simulink model "IEEE_34_node_2020a_scenarios"  (R2020a)
settings: Solver=FixedStepDiscrete  StartTime=0.0  StopTime=0.001  RelTol=1e-3
InitFcn:
  | power_34NodeTestFeeder_init;
  | %=============================
  | Vnom_ph_ph = 24900;
  | Vnom = 24900/sqrt(3);
  | Vnom1_ph_ph = 4160;
  | Vnom1 = 4160/sqrt(3);
  | Degrees_ph_ph_gen1 = 0;
  | Frequency = 60;
  | Apparent_power_gen1 = 2500e3;
  | base_current=1.5e6;
  | SW850_816=1;
  | SW818_820=1;
  | SW832_858=1;
  | SW834_842=1;
  | SW836_862=1;
  | %=============================
  | %824-828===Load1=================
  | V_824_828 = [1.008 1.016 1.012];
  | Pa_824_828 = [1e-6 1e-6 4]*1e3*1;
  | Pp_824_828 = [1e-6 1e-6 2]*1e3*1;
  | Pn_824_828 = [1e-6 1e-6 1e-6]*1;
  | 
  | %820-822===Load2=================
  | V_820_822 = 0.993;
  | Pa_820_822 = 135e3*1;
  | Pp_820_822 = 70e3*1;
  | Pn_820_822 = 1e-6*1;
  | 
  | %858-834===Load3=================
  | V_858_834 = [1.034 1.032 1.034]*sqrt(3);
  | Pa_858_834 = [4 15 13]*1e3*1;
  | Pp_858_834 = [2 8 7]*1e3*1;
  | Pn_858_834 = [1e-6 1e-6 1e-6]*1;
  | 
  | %844 B.V.c===Load4================
  | V_844 = [1.031 1.029 1.031];
  | Pa_844 = [135 135 135]*1e3*1;
  | Pp_844 = [105 105 105]*1e3*1;
  | Pn_844 = [100 100 100]*1e3*1;
  | 
  | %840======Load5=================
  | V_840 = [1.03 1.029 1.031];
  | Pa_840 = [9 9 9]*1e3*1;
  | Pp_840 = [7 7 7]*1e3*1;
  | Pn_840 = [1e-6 1e-6 1e-6]*1;
  | 
  | % For Distributed Loads==================================================
  | %802-806
  | V_802_806 = [1.047 1.048 1.048];
  | Pa_802_806 = [1e-6 30 25]*1e3;
  | Pp_802_806 = [1e-6 15 14]*1e3;
  | Pn_802_806 = [1e-6 1e-6 1e-6];
  | 
  | %808-810
  | V_808_810 = 1.014;
  | Pa_808_810 = 16e3;
  | Pp_808_810 = 8e3;
  | Pn_808_810 = 1e-6;
  | 
  | %816-824
  | V_816_824 = [1.017 1.025 1.02]*sqrt(3);
  | Pa_816_824 = [1e-6 5 1e-6]*1e3;
  | Pp_816_824 = [1e-6 2 1e-6]*1e3;
  | Pn_816_824 = [1e-6 1e-6 1e-6];
  | 
  | %818-820
  | V_818_820 = 1.016;
  | Pa_818_820 = 34e3;
  | Pp_818_820 = 17e3;
  | Pn_818_820 = 1e-6;
  | 
  | %824-826
  | V_824_826 = 1.008;
  | Pa_824_826 = 40e3;
  | Pp_824_826 = 20e3;
  | Pn_824_826 = 1e-6;
  | 
  | %828-830
  | V_828_830 = [1.007 1.015 1.011];
  | Pa_828_830 = [7 1e-6 1e-6]*1e3;
  | Pp_828_830 = [3 1e-6 1e-6]*1e3;
  | Pn_828_830 = [1e-6 1e-6 1e-6];
  | 
  | %832-858
  | V_832_858 = [1.036 1.035 1.036]*sqrt(3);
  | Pa_832_858 = [7 2 6]*1e3;
  | Pp_832_858 = [3 1 3]*1e3;
  | Pn_832_858 = [1e-6 1e-6 1e-6];
  | 
  | %834-860
  | V_834_860 = [1.031 1.029 1.031]*sqrt(3);
  | Pa_834_860 = [16 20 110]*1e3;
  | Pp_834_860 = [8 10 55]*1e3;
  | Pn_834_860 = [1e-6 1e-6 1e-6];
  | 
  | %836-840
  | V_836_840 = [1.03 1.029 1.031]*sqrt(3);
  | Pa_836_840 = [18 22 1e-6]*1e3;
  | Pp_836_840 = [9 11 1e-6]*1e3;
  | Pn_836_840 = [1e-6 1e-6 1e-6];
  | 
  | %842-844
  | V_842_844 = [1.031 1.029 1.031];
  | Pa_842_844 = [9 1e-6 1e-6]*1e3;
  | Pp_842_844 = [5 1e-6 1e-6]*1e3;
  | Pn_842_844 = [1e-6 1e-6 1e-6];
  | 
  | %844-846
  | V_844_846 = [1.031 1.029 1.031];
  | Pa_844_846 = [1e-6 25 20]*1e3;
  | Pp_844_846 = [1e-6 12 11]*1e3;
  | Pn_844_846 = [1e-6 1e-6 1e-6];
  | 
  | %846-848
  | V_846_848 = [1.031 1.029 1.031];
  | Pa_846_848 = [1e-6 23 1e-6]*1e3;
  | Pp_846_848 = [1e-6 11 1e-6]*1e3;
  | Pn_846_848 = [1e-6 1e-6 1e-6];
  | 
  | %854-856
  | V_854_856 = 0.998;
  | Pa_854_856 = 4e3;
  | Pp_854_856 = 2e3;
  | Pn_854_856 = 1e-6;
  | 
  | %858-864
  | V_858_864 = 1.034;
  | Pa_858_864 = 2e3;
  | Pp_858_864 = 1e3;
  | Pn_858_864 = 1e-6;
  | 
  | %860-836
  | V_860_836 = [1.03 1.029 1.031]*sqrt(3);
  | Pa_860_836 = [30 10 42]*1e3;
  | Pp_860_836 = [15 6 22]*1e3;
  | Pn_860_836 = [1e-6 1e-6 1e-6];
  | 
  | %862-838
  | V_862_838 = 1.029;
  | Pa_862_838 = 28e3;
  | Pp_862_838 = 14e3;
  | Pn_862_838 = 1e-6;
  | 
  | % For Spot Loads===========================================================
  | %830
  | V_830 = [0.989 0.998 0.994]*sqrt(3);
  | Pa_830 = [10 10 25]*1e3;
  | Pp_830 = [5 5 10]*1e3;
  | Pn_830 = [1e-6 1e-6 1e-6];
  | 
  | %848 B.V.c
  | V_848 = [1.031 1.029 1.031]*sqrt(3);
  | Pa_848 = [20 20 20]*1e3;
  | Pp_848 = [16 16 16]*1e3;
  | Pn_848 = [150 150 150]*1e3;
  | 
  | %860
  | V_860 = [1.03 1.029 1.031];
  | Pa_860 = [20 20 20]*1e3;
  | Pp_860 = [16 16 16]*1e3;
  | Pn_860 = [1e-6 1e-6 1e-6];
  | 
  | %890
  | V_890 = [0.917 0.924 0.918]*sqrt(3);
  | Pa_890 = [150 150 150]*1e3;
  | Pp_890 = [75 75 75]*1e3;
  | Pn_890 = [1e-6 1e-6 1e-6];
undefined symbols (not defined in the file or in its folder): Angle, C_300, C_301, C_302, C_303, C_304, Degrees_ph, ft2km, L_300, L_301, L_302, L_303, L_304, Magnitude, ph, ph_gen1, R_300, R_301, R_302, R_303, R_304, Vnom_ph
libraries: powerlib x177
(part 1 of 2)
settings Model: Creator=liyifu  LastModifiedBy=l4729
settings DataIOCC: ReturnWorkspaceOutputs=off
settings DebuggingCC: ArithmeticOperatorsInVariantConditions=warning
settings SFSimCC: SimUseLocalCustomCode=off  CustomCodeUndefinedFunction=UseInterfaceOnly
settings RTWCC: RTWUseLocalCustomCode=off

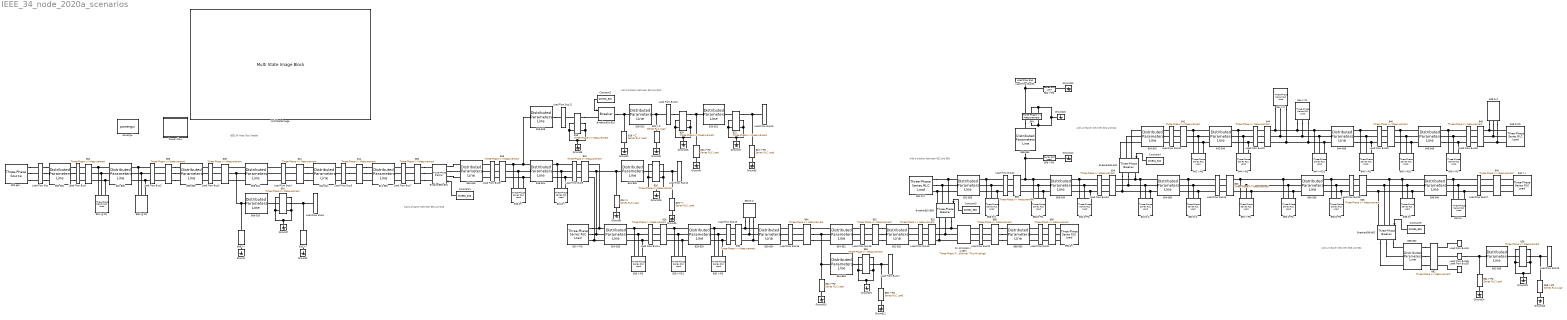
== system IEEE_34_node_2020a_scenarios ==
  note: Add a breaker between 832 and 858.
  note: IEEE 34 Node Test Feeder
  note: Add a breaker between 834 and 842.
  note: Add a breaker between 836 and 862.
  note: Add a breaker between 850 and 816.
  note: Add a breaker between 818 and 820.
  800 gen : powerlib/Electrical Sources/Three-Phase Source  InternalConnection=Yg  VoltagePhases=on  Voltage=Vnom_ph-ph  PhaseAngle=Degrees_ph-ph_gen1  Voltage_phases=[1.05 1.05 1.05]*Vnom  PhaseAngles_phases=[0 -120 +120]  Frequency=Frequency  NonIdealSource=off  SpecifyImpedance=on  Resistance=0.8929  Inductance=16.58e-3  ShortCircuitLevel=Apparent_power_gen1  BaseVoltage=Vnom_ph_ph  XRratio=8  BusType=swing  Pref=10e3  Qref=0  Prefabc=[10e3, 10e3, 10e3]  Qrefabc=[0, 0, 0]  Qmin=-inf  Qmax=inf
  800-802 : powerlib/Elements/Distributed Parameters Line  Phases=3  Frequency=Frequency  Resistance=R_300  Inductance=L_300  Capacitance=C_300  Length=2580*ft2km  x1=[1249.92108084395 26131.4308609001 26009.0181767455;376.991118430775 376.991118430775 376.991118430775;1.94160573810255 0.298080075052811 1.87234868535801]  x2=[1257.88413999223 26107.2604081607 25983.4031146893;376.991118430775 376.991118430775 376.991118430775;1.93808304381954 0.296564583820107 1.87075775483118]  x3=[7.14100156005761 32.3182501048481 23.0835619548769;376.991118430775 376.991118430775 376.991118430775;0.710958188620726 -0.81341186108836 0.253484207816933]  x4=[6.75597430008896 144.846280562991 132.525305942294;376.991118430775 376.991118430775 376.991118430775;-2.867320724315 0.497988283168986 2.04589027410211]  x5=3.46223763231864e-06  V1=ones(3,3)  V2=ones(3,3)  I1=ones(3,3)  I2=ones(3,3)  nHarmo=1  Measurements=None
  802 : powerlib/Measurements/Three-Phase V-I Measurement  VoltageMeasurement=phase-to-ground  SetLabelV=on  LabelV=Vabc_802  Vpu=on  VpuLL=off  CurrentMeasurement=yes  SetLabelI=on  LabelI=Iabc_802  Ipu=on  Pbase=base_current  Vbase=Vnom_ph_ph  OutputType=Magnitude-Angle  PhasorSimulation=on  PSBequivalent=0
  802 Yg PQ : powerlib/Elements/Three-Phase Series RLC Load  LConnTagsString=A|B|C  Configuration=Y (grounded)  NominalVoltage=[  Vabc=V_802_806*Vnom  Vabcp=[1e3 1e3 1e3]  NominalFrequency=Frequency  UnbalancedPower=on  ActivePower=10e3  InductivePower=100  CapacitivePower=100  Pabc=Pa_802_806/2  QLabc=Pp_802_806/2  QCabc=Pn_802_806  Pabcp=[10e3 9e3 11e3]  QLabcp=[100 90 110]  QCabcp=[100 90 110]  Measurements=None  LoadType=constant PQ
      settings: AttributesFormatString=|
      | P= %<Pabc> W
      | Ql=%<QLabc> var
      | Qc=%<QCabc> var
  802-806 : powerlib/Elements/Distributed Parameters Line  Phases=3  Frequency=Frequency  Resistance=R_300  Inductance=L_300  Capacitance=C_300  Length=1730*ft2km  x1=[1257.88413999223 26107.2604081607 25983.4031146893;376.991118430775 376.991118430775 376.991118430775;1.93851306238997 0.296931084446931 1.87111711923874]  x2=[1263.03152773622 26091.3668630639 25967.0505546349;376.991118430775 376.991118430775 376.991118430775;1.93675476604224 0.29592284444399 1.87004699504629]  x3=[6.74174515393169 32.6757565944536 24.2819591482835;376.991118430775 376.991118430775 376.991118430775;0.818712189904275 -0.791719291330259 0.305405947950471]  x4=[6.06467042248893 143.993748432463 131.480607437597;376.991118430775 376.991118430775 376.991118430775;-2.79230394021469 0.498395409094565 2.05596025477108]  x5=2.32157794725242e-06  V1=ones(3,3)  V2=ones(3,3)  I1=ones(3,3)  I2=ones(3,3)  nHarmo=1  Measurements=None
  806 : powerlib/Measurements/Three-Phase V-I Measurement  VoltageMeasurement=phase-to-ground  SetLabelV=on  LabelV=Vabc_806  Vpu=on  VpuLL=off  CurrentMeasurement=yes  SetLabelI=on  LabelI=Iabc_806  Ipu=on  Pbase=base_current  Vbase=Vnom_ph_ph  OutputType=Magnitude-Angle  PhasorSimulation=on  PSBequivalent=0
  806 Yg PQ : powerlib/Elements/Three-Phase Series RLC Load  LConnTagsString=A|B|C  Configuration=Y (grounded)  NominalVoltage=[  Vabc=V_802_806*Vnom  Vabcp=[1e3 1e3 1e3]  NominalFrequency=Frequency  UnbalancedPower=on  ActivePower=10e3  InductivePower=100  CapacitivePower=100  Pabc=Pa_802_806/2  QLabc=Pp_802_806/2  QCabc=Pn_802_806  Pabcp=[10e3 9e3 11e3]  QLabcp=[100 90 110]  QCabcp=[100 90 110]  Measurements=None  LoadType=constant PQ
      settings: AttributesFormatString=|
      | P= %<Pabc> W
      | Ql=%<QLabc> var
      | Qc=%<QCabc> var
  806-808 : powerlib/Elements/Distributed Parameters Line  Phases=3  Frequency=Frequency  Resistance=R_300  Inductance=L_300  Capacitance=C_300  Length=32230*ft2km  x1=[1263.03152773622 26091.3668630639 25967.0505546349;376.991118430775 376.991118430775 376.991118430775;1.9213246879271 0.282771939599148 1.85715215453986]  x2=[1355.36741013163 25802.965279815 25680.3228944133;376.991118430775 376.991118430775 376.991118430775;1.90106006488918 0.264077284558239 1.83705579461531]  x3=[6.38688498732981 32.5400387220186 25.3091222711061;376.991118430775 376.991118430775 376.991118430775;0.921699027337811 -0.793519160961749 0.32962763678599]  x4=[5.32362115475156 140.079806740904 128.071939191277;376.991118430775 376.991118430775 376.991118430775;-2.73237240417034 0.470552224502591 2.03887968104344]  x5=4.32511313525697e-05  V1=ones(3,3)  V2=ones(3,3)  I1=ones(3,3)  I2=ones(3,3)  nHarmo=1  Measurements=None
  808 : powerlib/Measurements/Three-Phase V-I Measurement  VoltageMeasurement=phase-to-ground  SetLabelV=on  LabelV=Vabc_808  Vpu=on  VpuLL=off  CurrentMeasurement=yes  SetLabelI=on  LabelI=Iabc_808  Ipu=on  Pbase=base_current  Vbase=Vnom_ph_ph  OutputType=Magnitude-Angle  PhasorSimulation=on  PSBequivalent=0
  808 Y-I : powerlib/Elements/Series RLC Load  LConnTagsString=a  RConnTagsString=__new0  NominalVoltage=V_808_810*Vnom  NominalFrequency=Frequency  ActivePower=Pa_808_810/2  InductivePower=Pp_808_810/2  CapacitivePower=Pn_808_810  Setx0=off  InitialVoltage=0  SetiL0=off  InitialCurrent=0  Measurements=None  LoadType=constant I
      settings: AttributesFormatString=|
      | P=%<ActivePower> W
      | Ql=%<InductivePower> var
      | Qc=%<CapacitivePower> var
  808-810 : powerlib/Elements/Distributed Parameters Line  Phases=1  Frequency=Frequency  Resistance=R_303(2,2)  Inductance=L_303(2,2)  Capacitance=C_303(2,2)  Length=5804*ft2km  x1=[21046.9259463273;376.991118430775;-2.12176175592429]  x2=[21043.9208768996;376.991118430775;-2.12177244967677]  x3=[34.5685211736535;376.991118430775;-2.11315216164077]  x4=[36.1447450908434;376.991118430775;-2.13270369941523]  x5=7.30496713110932e-06  V1=ones(3,3)  V2=ones(3,3)  I1=ones(3,3)  I2=ones(3,3)  nHarmo=1  Measurements=None
  808-812 : powerlib/Elements/Distributed Parameters Line  Phases=3  Frequency=Frequency  Resistance=R_300  Inductance=L_300  Capacitance=C_300  Length=37500*ft2km  x1=[1355.36741013163 25802.965279815 25680.3228944133;376.991118430775 376.991118430775 376.991118430775;1.89839394975256 0.261804980671934 1.83482773528846]  x2=[1443.84439604931 25478.3634476897 25362.7536549307;376.991118430775 376.991118430775 376.991118430775;1.88315754512085 0.240205062784278 1.81096458108983]  x3=[5.47970534503738 32.5458510221011 26.6156539334698;376.991118430775 376.991118430775 376.991118430775;0.996384506820799 -0.794758877830925 0.308471950569626]  x4=[4.24120551746674 137.246147529385 126.440066991532;376.991118430775 376.991118430775 376.991118430775;-2.80340516655793 0.448617182172184 2.02664641407674]  x5=5.03232213999802e-05  V1=ones(3,3)  V2=ones(3,3)  I1=ones(3,3)  I2=ones(3,3)  nHarmo=1  Measurements=None
  810 : powerlib/Measurements/Three-Phase V-I Measurement  VoltageMeasurement=phase-to-ground  SetLabelV=on  LabelV=Vabc_810  Vpu=on  VpuLL=off  CurrentMeasurement=yes  SetLabelI=on  LabelI=Iabc_810  Ipu=on  Pbase=base_current  Vbase=Vnom_ph_ph  OutputType=Magnitude-Angle  PhasorSimulation=on  PSBequivalent=0
  810 Y-I : powerlib/Elements/Series RLC Load  LConnTagsString=a  RConnTagsString=__new0  NominalVoltage=V_808_810*Vnom  NominalFrequency=Frequency  ActivePower=Pa_808_810/2  InductivePower=Pp_808_810/2  CapacitivePower=Pn_808_810  Setx0=off  InitialVoltage=0  SetiL0=off  InitialCurrent=0  Measurements=None  LoadType=constant I
      settings: AttributesFormatString=|
      | P=%<ActivePower> W
      | Ql=%<InductivePower> var
      | Qc=%<CapacitivePower> var
  812 : powerlib/Measurements/Three-Phase V-I Measurement  VoltageMeasurement=phase-to-ground  SetLabelV=on  LabelV=Vabc_812  Vpu=on  VpuLL=off  CurrentMeasurement=yes  SetLabelI=on  LabelI=Iabc_812  Ipu=on  Pbase=base_current  Vbase=Vnom_ph_ph  OutputType=Magnitude-Angle  PhasorSimulation=on  PSBequivalent=0
  812-814 : powerlib/Elements/Distributed Parameters Line  Phases=3  Frequency=Frequency  Resistance=R_300  Inductance=L_300  Capacitance=C_300  Length=29730*ft2km  x1=[1443.84439604931 25478.3634476897 25362.7536549307;376.991118430775 376.991118430775 376.991118430775;1.88708842075871 0.243555309690653 1.81424959455655]  x2=[1513.83129923695 25224.7890628026 25116.826082141;376.991118430775 376.991118430775 376.991118430775;1.87645290964613 0.226315237464506 1.79513044997697]  x3=[5.55063231072111 32.5564691162332 27.1376298044207;376.991118430775 376.991118430775 376.991118430775;1.01612398171474 -0.820636608900659 0.284298301573858]  x4=[4.1999268951778 136.474072334335 125.741278014505;376.991118430775 376.991118430775 376.991118430775;-2.81942996147556 0.43687198855717 2.01560545263332]  x5=3.98962499259043e-05  V1=ones(3,3)  V2=ones(3,3)  I1=ones(3,3)  I2=ones(3,3)  nHarmo=1  Measurements=None
  814 : powerlib/Measurements/Three-Phase V-I Measurement  VoltageMeasurement=phase-to-ground  SetLabelV=on  LabelV=Vabc_814  Vpu=on  VpuLL=off  CurrentMeasurement=yes  SetLabelI=on  LabelI=Iabc_814  Ipu=on  Pbase=base_current  Vbase=Vnom_ph_ph  OutputType=Magnitude-Angle  PhasorSimulation=on  PSBequivalent=0
  814-850 : powerlib/Elements/Distributed Parameters Line  Phases=3  Frequency=Frequency  Resistance=R_301  Inductance=L_301  Capacitance=C_301  Length=10*ft2km  x1=[749.15329467254 25227.0261178494 25140.714564817;376.991118430775 376.991118430775 376.991118430775;-0.62406898031134 0.237616780416975 1.80414776598586]  x2=[749.130082958643 25226.8770754942 25140.5688252729;376.991118430775 376.991118430775 376.991118430775;-0.624045610021532 0.237609694611455 1.80414003880896]  x3=[4.47496846801465 31.8833259534658 28.1266540016917;376.991118430775 376.991118430775 376.991118430775;0.864239655329809 -0.885362952079534 0.234866042830331]  x4=[4.63631302404033 136.170219123993 125.22263936746;376.991118430775 376.991118430775 376.991118430775;-1.91799176304395 0.450265085785532 2.03068759542421]  x5=1.37899021776565e-08  V1=ones(3,3)  V2=ones(3,3)  I1=ones(3,3)  I2=ones(3,3)  nHarmo=1  Measurements=None
  816 : powerlib/Measurements/Three-Phase V-I Measurement  VoltageMeasurement=phase-to-ground  SetLabelV=on  LabelV=Vabc_816  Vpu=on  VpuLL=off  CurrentMeasurement=yes  SetLabelI=on  LabelI=Iabc_816  Ipu=on  Pbase=base_current  Vbase=Vnom_ph_ph  OutputType=Magnitude-Angle  PhasorSimulation=on  PSBequivalent=0
  816 D-I : powerlib/Elements/Three-Phase Series RLC Load  LConnTagsString=A|B|C  Configuration=Delta  NominalVoltage=[  Vabc=[1.017 1.025 1.02]*sqrt(3)*Vnom  Vabcp=V_816_824*Vnom  NominalFrequency=Frequency  UnbalancedPower=on  ActivePower=10e3  InductivePower=100  CapacitivePower=100  Pabc=[0 30 25]*1e3/2  QLabc=[0 15 14]*1e3/2  QCabc=[0 0 0]  Pabcp=Pa_816_824/2  QLabcp=Pp_816_824/2  QCabcp=Pn_816_824  Measurements=None  LoadType=constant I
      settings: AttributesFormatString=|
      | P= %<Pabc> W
      | Ql=%<QLabc> var
      | Qc=%<QCabc> var
  816-818 : powerlib/Elements/Distributed Parameters Line  Phases=1  Frequency=Frequency  Resistance=R_302(1,1)  Inductance=L_302(1,1)  Capacitance=C_302(1,1)  Length=1710*ft2km  x1=[20490.3042148397;376.991118430775;-0.0532544135280046]  x2=[20490.3109594136;376.991118430775;-0.053255033845596]  x3=[34.5169728301595;376.991118430775;-0.0540660920901116]  x4=[34.5169728344743;376.991118430775;-0.0532550338463431]  x5=2.15222153587128e-06  V1=ones(3,3)  V2=ones(3,3)  I1=ones(3,3)  I2=ones(3,3)  nHarmo=1  Measurements=None
  816-824 : powerlib/Elements/Distributed Parameters Line  Phases=3  Frequency=Frequency  Resistance=R_301  Inductance=L_301  Capacitance=C_301  Length=10210*ft2km  x1=[748.410739748618 25222.2511977151 25136.0453810114;376.991118430775 376.991118430775 376.991118430775;-0.628622488455534 0.233068321988764 1.79964654831585]  x2=[724.867335226711 25070.57527146 24988.5436693509;376.991118430775 376.991118430775 376.991118430775;-0.603933885970706 0.225820727896608 1.79171985964701]  x3=[4.47046107178887 31.6153299611701 28.1466881681829;376.991118430775 376.991118430775 376.991118430775;0.861223606040793 -0.892893782392515 0.231267715388187]  x4=[4.61080299055656 134.671592338258 123.966064883203;376.991118430775 376.991118430775 376.991118430775;-1.92687304548077 0.440217730369648 2.02260235021295]  x5=1.40794901233873e-05  V1=ones(3,3)  V2=ones(3,3)  I1=ones(3,3)  I2=ones(3,3)  nHarmo=1  Measurements=None
  818 : powerlib/Measurements/Three-Phase V-I Measurement  VoltageMeasurement=phase-to-ground  SetLabelV=on  LabelV=Vabc_818  Vpu=on  VpuLL=off  CurrentMeasurement=yes  SetLabelI=on  LabelI=Iabc_818  Ipu=on  Pbase=base_current  Vbase=Vnom_ph_ph  OutputType=Magnitude-Angle  PhasorSimulation=on  PSBequivalent=0
  818 Y-Z : powerlib/Elements/Series RLC Load  LConnTagsString=a  RConnTagsString=__new0  NominalVoltage=V_818_820*Vnom  NominalFrequency=Frequency  ActivePower=Pa_818_820/2  InductivePower=Pp_818_820/2  CapacitivePower=Pn_818_820  Setx0=off  InitialVoltage=0  SetiL0=off  InitialCurrent=0  Measurements=None  LoadType=constant Z
      settings: AttributesFormatString=|
      | P=%<ActivePower> W
      | Ql=%<InductivePower> var
      | Qc=%<CapacitivePower> var
  818-820 : powerlib/Elements/Distributed Parameters Line  Phases=1  Frequency=Frequency  Resistance=R_302(1,1)  Inductance=L_302(1,1)  Capacitance=C_302(1,1)  Length=48150*ft2km  x1=[2.78170730011638e-10;376.991118430775;-2.73913993190896]  x2=[2.75226069334982e-10;376.991118430775;-2.713474091581]  x3=[5.39302235223237e-13;376.991118430775;-2.24824250678969]  x4=[4.97303653528767e-13;376.991118430775;3.01000433404245]  x5=6.06020274574283e-05  V1=ones(3,3)  V2=ones(3,3)  I1=ones(3,3)  I2=ones(3,3)  nHarmo=1  Measurements=None
  820 : powerlib/Measurements/Three-Phase V-I Measurement  VoltageMeasurement=phase-to-ground  SetLabelV=on  LabelV=Vabc_820  Vpu=on  VpuLL=off  CurrentMeasurement=yes  SetLabelI=on  LabelI=Iabc_820  Ipu=on  Pbase=base_current  Vbase=Vnom_ph_ph  OutputType=Magnitude-Angle  PhasorSimulation=on  PSBequivalent=0
  820 Y-PQ : powerlib/Elements/Series RLC Load  LConnTagsString=a  RConnTagsString=__new0  NominalVoltage=V_820_822*Vnom  NominalFrequency=Frequency  ActivePower=Pa_820_822/2  InductivePower=Pp_820_822/2  CapacitivePower=Pn_820_822  Setx0=off  InitialVoltage=0  SetiL0=off  InitialCurrent=0  Measurements=None  LoadType=constant PQ
      settings: AttributesFormatString=|
      | P=%<ActivePower> W
      | Ql=%<InductivePower> var
      | Qc=%<CapacitivePower> var
  820 Y-Z : powerlib/Elements/Series RLC Load  LConnTagsString=a  RConnTagsString=__new0  NominalVoltage=V_818_820*Vnom  NominalFrequency=Frequency  ActivePower=Pa_818_820/2  InductivePower=Pp_818_820/2  CapacitivePower=Pn_818_820  Setx0=off  InitialVoltage=0  SetiL0=off  InitialCurrent=0  Measurements=None  LoadType=constant Z
      settings: AttributesFormatString=|
      | P=%<ActivePower> W
      | Ql=%<InductivePower> var
      | Qc=%<CapacitivePower> var
  820-822 : powerlib/Elements/Distributed Parameters Line  Phases=1  Frequency=Frequency  Resistance=R_302(1,1)  Inductance=L_302(1,1)  Capacitance=C_302(1,1)  Length=13740*ft2km  x1=[2.75226069334982e-10;376.991118430775;-2.69714708176881]  x2=[2.74353965241595e-10;376.991118430775;-2.69721735196413]  x3=[3.68825505705946e-13;376.991118430775;-2.57289838354741]  x4=[5.5452475643169e-13;376.991118430775;-2.78516167237058]  x5=1.72932888320886e-05  V1=ones(3,3)  V2=ones(3,3)  I1=ones(3,3)  I2=ones(3,3)  nHarmo=1  Measurements=None
  822 : powerlib/Measurements/Three-Phase V-I Measurement  VoltageMeasurement=phase-to-ground  SetLabelV=on  LabelV=Vabc_822  Vpu=on  VpuLL=off  CurrentMeasurement=yes  SetLabelI=on  LabelI=Iabc_822  Ipu=on  Pbase=base_current  Vbase=Vnom_ph_ph  OutputType=Magnitude-Angle  PhasorSimulation=on  PSBequivalent=0
  822 Y-PQ : powerlib/Elements/Series RLC Load  LConnTagsString=a  RConnTagsString=__new0  NominalVoltage=V_820_822*Vnom  NominalFrequency=Frequency  ActivePower=Pa_820_822/2  InductivePower=Pp_820_822/2  CapacitivePower=Pn_820_822  Setx0=off  InitialVoltage=0  SetiL0=off  InitialCurrent=0  Measurements=None  LoadType=constant PQ
      settings: AttributesFormatString=|
      | P=%<ActivePower> W
      | Ql=%<InductivePower> var
      | Qc=%<CapacitivePower> var
  824 : powerlib/Measurements/Three-Phase V-I Measurement  VoltageMeasurement=phase-to-ground  SetLabelV=on  LabelV=Vabc_824  Vpu=on  VpuLL=off  CurrentMeasurement=yes  SetLabelI=on  LabelI=Iabc_824  Ipu=on  Pbase=base_current  Vbase=Vnom_ph_ph  OutputType=Magnitude-Angle  PhasorSimulation=on  PSBequivalent=0
  824 D-I : powerlib/Elements/Three-Phase Series RLC Load  LConnTagsString=A|B|C  Configuration=Delta  NominalVoltage=[  Vabc=[1.017 1.025 1.02]*sqrt(3)*Vnom  Vabcp=V_816_824*Vnom  NominalFrequency=Frequency  UnbalancedPower=on  ActivePower=10e3  InductivePower=100  CapacitivePower=100  Pabc=[0 30 25]*1e3/2  QLabc=[0 15 14]*1e3/2  QCabc=[0 0 0]  Pabcp=Pa_816_824/2  QLabcp=Pp_816_824/2  QCabcp=Pn_816_824  Measurements=None  LoadType=constant I
      settings: AttributesFormatString=|
      | P= %<Pabc> W
      | Ql=%<QLabc> var
      | Qc=%<QCabc> var
  824 Y-I : powerlib/Elements/Series RLC Load  LConnTagsString=a  RConnTagsString=__new0  NominalVoltage=V_824_826*Vnom  NominalFrequency=Frequency  ActivePower=Pa_824_826/2  InductivePower=Pp_824_826/2  CapacitivePower=Pn_824_826  Setx0=off  InitialVoltage=0  SetiL0=off  InitialCurrent=0  Measurements=None  LoadType=constant I
      settings: AttributesFormatString=|
      | P=%<ActivePower> W
      | Ql=%<InductivePower> var
      | Qc=%<CapacitivePower> var
  824 Y-PQ : powerlib/Elements/Three-Phase Series RLC Load  LConnTagsString=A|B|C  Configuration=Y (grounded)  NominalVoltage=[  Vabc=V_824_828*Vnom  Vabcp=[1.008 1.016 1.012]*Vnom  NominalFrequency=Frequency  UnbalancedPower=on  ActivePower=10e3  InductivePower=100  CapacitivePower=100  Pabc=Pa_824_828/2  QLabc=Pp_824_828/2  QCabc=Pn_824_828  Pabcp=[0 0 4]*1e3/2  QLabcp=[0 0 2]*1e3/2  QCabcp=[0 0 0]  Measurements=None  LoadType=constant PQ
      settings: AttributesFormatString=|
      | P= %<Pabc> W
      | Ql=%<QLabc> var
      | Qc=%<QCabc> var
  824-826 : powerlib/Elements/Distributed Parameters Line  Phases=1  Frequency=Frequency  Resistance=R_303(2,2)  Inductance=L_303(2,2)  Capacitance=C_303(2,2)  Length=3030*ft2km  x1=[20429.4672255499;376.991118430775;-2.17401307078524]  x2=[20425.5338147724;376.991118430775;-2.17401970407193]  x3=[32.4543868781171;376.991118430775;-2.14560246141602]  x4=[36.3331475022774;376.991118430775;-2.20075809708011]  x5=3.81358552847368e-06  V1=ones(3,3)  V2=ones(3,3)  I1=ones(3,3)  I2=ones(3,3)  nHarmo=1  Measurements=None
  824-828 : powerlib/Elements/Distributed Parameters Line  Phases=3  Frequency=Frequency  Resistance=R_301  Inductance=L_301  Capacitance=C_301  Length=840*ft2km  x1=[724.867335226711 25070.57527146 24988.5436693509;376.991118430775 376.991118430775 376.991118430775;-0.599062731576336 0.229790647439184 1.79562752415418]  x2=[723.397409454072 25058.7323545982 24977.0680880783;376.991118430775 376.991118430775 376.991118430775;-0.598766489746599 0.229212934219949 1.79495279123407]  x3=[2.36923914486667 32.3485909598067 30.8832169996217;376.991118430775 376.991118430775 376.991118430775;1.29473424498697 -0.817995484780134 0.258235979195186]  x4=[3.23899011357272 132.699107328167 124.093614434081;376.991118430775 376.991118430775 376.991118430775;-1.3656517787228 0.44205405107672 2.04648096663621]  x5=1.15835178292315e-06  V1=ones(3,3)  V2=ones(3,3)  I1=ones(3,3)  I2=ones(3,3)  nHarmo=1  Measurements=None
  826 : powerlib/Measurements/Three-Phase V-I Measurement  VoltageMeasurement=phase-to-ground  SetLabelV=on  LabelV=Vabc_826  Vpu=on  VpuLL=off  CurrentMeasurement=yes  SetLabelI=on  LabelI=Iabc_826  Ipu=on  Pbase=base_current  Vbase=Vnom_ph_ph  OutputType=Magnitude-Angle  PhasorSimulation=on  PSBequivalent=0
  826 Y-I : powerlib/Elements/Series RLC Load  LConnTagsString=a  RConnTagsString=__new0  NominalVoltage=V_824_826*Vnom  NominalFrequency=Frequency  ActivePower=Pa_824_826/2  InductivePower=Pp_824_826/2  CapacitivePower=Pn_824_826  Setx0=off  InitialVoltage=0  SetiL0=off  InitialCurrent=0  Measurements=None  LoadType=constant I
      settings: AttributesFormatString=|
      | P=%<ActivePower> W
      | Ql=%<InductivePower> var
      | Qc=%<CapacitivePower> var
  828 : powerlib/Measurements/Three-Phase V-I Measurement  VoltageMeasurement=phase-to-ground  SetLabelV=on  LabelV=Vabc_828  Vpu=on  VpuLL=off  CurrentMeasurement=yes  SetLabelI=on  LabelI=Iabc_828  Ipu=on  Pbase=base_current  Vbase=Vnom_ph_ph  OutputType=Magnitude-Angle  PhasorSimulation=on  PSBequivalent=0
  828 Y-PQ : powerlib/Elements/Three-Phase Series RLC Load  LConnTagsString=A|B|C  Configuration=Y (grounded)  NominalVoltage=[  Vabc=V_824_828*Vnom  Vabcp=[1.008 1.016 1.012]*Vnom  NominalFrequency=Frequency  UnbalancedPower=on  ActivePower=10e3  InductivePower=100  CapacitivePower=100  Pabc=Pa_824_828/2  QLabc=Pp_824_828/2  QCabc=Pn_824_828  Pabcp=[0 0 4]*1e3/2  QLabcp=[0 0 2]*1e3/2  QCabcp=[0 0 0]  Measurements=None  LoadType=constant PQ
      settings: AttributesFormatString=|
      | P= %<Pabc> W
      | Ql=%<QLabc> var
      | Qc=%<QCabc> var
  828 Y-PQ1 : powerlib/Elements/Three-Phase Series RLC Load  LConnTagsString=A|B|C  Configuration=Y (grounded)  NominalVoltage=[  Vabc=V_828_830*Vnom  Vabcp=[1.008 1.016 1.012]*Vnom  NominalFrequency=Frequency  UnbalancedPower=on  ActivePower=10e3  InductivePower=100  CapacitivePower=100  Pabc=Pa_828_830/2  QLabc=Pp_828_830/2  QCabc=Pn_828_830  Pabcp=[0 0 4]*1e3/2  QLabcp=[0 0 2]*1e3/2  QCabcp=[0 0 0]  Measurements=None  LoadType=constant PQ
      settings: AttributesFormatString=|
      | P= %<Pabc> W
      | Ql=%<QLabc> var
      | Qc=%<QCabc> var
  828-830 : powerlib/Elements/Distributed Parameters Line  Phases=3  Frequency=Frequency  Resistance=R_301  Inductance=L_301  Capacitance=C_301  Length=20440*ft2km  x1=[723.397409454072 25058.7323545982 24977.0680880783;376.991118430775 376.991118430775 376.991118430775;-0.60895588421081 0.220908726852342 1.78677880784661]  x2=[687.890008443739 24774.2004000743 24701.7282543147;376.991118430775 376.991118430775 376.991118430775;-0.597379057690305 0.206735904708081 1.77027628259819]  x3=[2.432969435861 32.1805315871596 30.6464261998804;376.991118430775 376.991118430775 376.991118430775;1.20657377086038 -0.834137845152898 0.248764024490916]  x4=[3.17186158439525 129.86700661184 121.708708747769;376.991118430775 376.991118430775 376.991118430775;-1.44805057910995 0.425340619102156 2.02856900599009]  x5=2.81865600511299e-05  V1=ones(3,3)  V2=ones(3,3)  I1=ones(3,3)  I2=ones(3,3)  nHarmo=1  Measurements=None
  830 : powerlib/Measurements/Three-Phase V-I Measurement  VoltageMeasurement=phase-to-ground  SetLabelV=on  LabelV=Vabc_830  Vpu=on  VpuLL=off  CurrentMeasurement=yes  SetLabelI=on  LabelI=Iabc_830  Ipu=on  Pbase=base_current  Vbase=Vnom_ph_ph  OutputType=Magnitude-Angle  PhasorSimulation=on  PSBequivalent=0
  830 D-Z : powerlib/Elements/Three-Phase Series RLC Load  LConnTagsString=A|B|C  Configuration=Delta  NominalVoltage=[  Vabc=[1.017 1.025 1.02]*sqrt(3)*Vnom  Vabcp=V_830*Vnom  NominalFrequency=Frequency  UnbalancedPower=on  ActivePower=10e3  InductivePower=100  CapacitivePower=100  Pabc=[0 30 25]*1e3/2  QLabc=[0 15 14]*1e3/2  QCabc=[0 0 0]  Pabcp=Pa_830  QLabcp=Pp_830  QCabcp=Pn_830  Measurements=None  LoadType=constant Z
      settings: AttributesFormatString=|
      | P= %<Pabc> W
      | Ql=%<QLabc> var
      | Qc=%<QCabc> var
  830 Y-PQ : powerlib/Elements/Three-Phase Series RLC Load  LConnTagsString=A|B|C  Configuration=Y (grounded)  NominalVoltage=[  Vabc=V_828_830*Vnom  Vabcp=[1.008 1.016 1.012]*Vnom  NominalFrequency=Frequency  UnbalancedPower=on  ActivePower=10e3  InductivePower=100  CapacitivePower=100  Pabc=Pa_828_830/2  QLabc=Pp_828_830/2  QCabc=Pn_828_830  Pabcp=[0 0 4]*1e3/2  QLabcp=[0 0 2]*1e3/2  QCabcp=[0 0 0]  Measurements=None  LoadType=constant PQ
      settings: AttributesFormatString=|
      | P= %<Pabc> W
      | Ql=%<QLabc> var
      | Qc=%<QCabc> var
  830-854 : powerlib/Elements/Distributed Parameters Line  Phases=3  Frequency=Frequency  Resistance=R_301  Inductance=L_301  Capacitance=C_301  Length=520*ft2km  x1=[687.890008443739 24774.2004000743 24701.7282543147;376.991118430775 376.991118430775 376.991118430775;-0.587023305765453 0.215175690971486 1.77858371877566]  x2=[687.074296441229 24767.4205301758 24695.151726903;376.991118430775 376.991118430775 376.991118430775;-0.586608473126875 0.21480794966191 1.77816745817774]  x3=[2.36435240131937 34.8453273283256 31.6473726025582;376.991118430775 376.991118430775 376.991118430775;1.09875282733498 -0.822065542458938 0.309079407862657]  x4=[2.94233840749575 129.978408735007 120.846503209265;376.991118430775 376.991118430775 376.991118430775;-1.51135724515578 0.447763697300477 2.04183833920304]  x5=7.17074913238139e-07  V1=ones(3,3)  V2=ones(3,3)  I1=ones(3,3)  I2=ones(3,3)  nHarmo=1  Measurements=None
  832 : powerlib/Measurements/Three-Phase V-I Measurement  VoltageMeasurement=phase-to-ground  SetLabelV=on  LabelV=Vabc_832  Vpu=on  VpuLL=off  CurrentMeasurement=yes  SetLabelI=on  LabelI=Iabc_832  Ipu=on  Pbase=base_current  Vbase=Vnom_ph_ph  OutputType=Magnitude-Angle  PhasorSimulation=on  PSBequivalent=0
  832 D-Z : powerlib/Elements/Three-Phase Series RLC Load  LConnTagsString=A|B|C  Configuration=Delta  NominalVoltage=[  Vabc=[1.017 1.025 1.02]*sqrt(3)*Vnom  Vabcp=V_832_858*Vnom  NominalFrequency=Frequency  UnbalancedPower=on  ActivePower=10e3  InductivePower=100  CapacitivePower=100  Pabc=[0 30 25]*1e3/2  QLabc=[0 15 14]*1e3/2  QCabc=[0 0 0]  Pabcp=Pa_832_858/2  QLabcp=Pp_832_858/2  QCabcp=Pn_832_858  Measurements=None  LoadType=constant Z
      settings: AttributesFormatString=|
      | P= %<Pabc> W
      | Ql=%<QLabc> var
      | Qc=%<QCabc> var
  832-858 : powerlib/Elements/Distributed Parameters Line  Phases=3  Frequency=Frequency  Resistance=R_301  Inductance=L_301  Capacitance=C_301  Length=4900*ft2km  x1=[635.221951350746 24292.4598320497 24240.3589940589;376.991118430775 376.991118430775 376.991118430775;-0.560180195954398 0.186796264913495 1.74652281231025]  x2=[631.73772567187 24266.2453880144 24217.7971104675;376.991118430775 376.991118430775 376.991118430775;-0.55639130492122 0.183171001314221 1.74249003415027]  x3=[1.40655489057687 53.5769646057378 47.4153326896052;376.991118430775 376.991118430775 376.991118430775;0.647268705057357 -0.659975964439056 0.640697617253904]  x4=[1.58197127828822 112.657712920708 104.837182641463;376.991118430775 376.991118430775 376.991118430775;-1.54023944511965 0.547259740334444 2.15897850543274]  x5=6.7570520670517e-06  V1=ones(3,3)  V2=ones(3,3)  I1=ones(3,3)  I2=ones(3,3)  nHarmo=1  Measurements=None
  834 : powerlib/Measurements/Three-Phase V-I Measurement  VoltageMeasurement=phase-to-ground  SetLabelV=on  LabelV=Vabc_834  Vpu=on  VpuLL=off  CurrentMeasurement=yes  SetLabelI=on  LabelI=Iabc_834  Ipu=on  Pbase=base_current  Vbase=Vnom_ph_ph  OutputType=Magnitude-Angle  PhasorSimulation=on  PSBequivalent=0
  834 D-PQ : powerlib/Elements/Three-Phase Series RLC Load  LConnTagsString=A|B|C  Configuration=Delta  NominalVoltage=[  Vabc=[1.017 1.025 1.02]*sqrt(3)*Vnom  Vabcp=V_858_834*Vnom  NominalFrequency=Frequency  UnbalancedPower=on  ActivePower=10e3  InductivePower=100  CapacitivePower=100  Pabc=[0 30 25]*1e3/2  QLabc=[0 15 14]*1e3/2  QCabc=[0 0 0]  Pabcp=Pa_858_834/2  QLabcp=Pp_858_834/2  QCabcp=Pn_858_834  Measurements=None  LoadType=constant PQ
      settings: AttributesFormatString=|
      | P= %<Pabc> W
      | Ql=%<QLabc> var
      | Qc=%<QCabc> var
  834 D-Z : powerlib/Elements/Three-Phase Series RLC Load  LConnTagsString=A|B|C  Configuration=Delta  NominalVoltage=[  Vabc=[1.017 1.025 1.02]*sqrt(3)*Vnom  Vabcp=V_834_860*Vnom  NominalFrequency=Frequency  UnbalancedPower=on  ActivePower=10e3  InductivePower=100  CapacitivePower=100  Pabc=[0 30 25]*1e3/2  QLabc=[0 15 14]*1e3/2  QCabc=[0 0 0]  Pabcp=Pa_834_860/2  QLabcp=Pp_834_860/2  QCabcp=Pn_834_860  Measurements=None  LoadType=constant Z
      settings: AttributesFormatString=|
      | P= %<Pabc> W
      | Ql=%<QLabc> var
      | Qc=%<QCabc> var
  834-842 : powerlib/Elements/Distributed Parameters Line  Phases=3  Frequency=Frequency  Resistance=R_301  Inductance=L_301  Capacitance=C_301  Length=280*ft2km  x1=[628.077515737555 24237.3294599899 24193.6526229152;376.991118430775 376.991118430775 376.991118430775;-0.548895046586725 0.180804935703686 1.73963207578974]  x2=[628.151716180336 24237.5914731138 24194.2083063583;376.991118430775 376.991118430775 376.991118430775;-0.549093747437041 0.180580768540891 1.73941288211016]  x3=[0.893365861338146 71.7600738793581 62.1788798857537;376.991118430775 376.991118430775 376.991118430775;-1.58038350095508 -0.616633004293201 0.839946272487654]  x4=[1.19184823205198 104.469274645666 92.6077704662745;376.991118430775 376.991118430775 376.991118430775;0.149482010807848 0.694379165632413 2.29305064846154]  x5=3.86117260974383e-07  V1=ones(3,3)  V2=ones(3,3)  I1=ones(3,3)  I2=ones(3,3)  nHarmo=1  Measurements=None
  834-860 : powerlib/Elements/Distributed Parameters Line  Phases=3  Frequency=Frequency  Resistance=R_301  Inductance=L_301  Capacitance=C_301  Length=2020*ft2km  x1=[628.077484124564 24237.3315138492 24193.654603702;376.991118430775 376.991118430775 376.991118430775;-0.549799527071236 0.180067937065794 1.73890662630872]  x2=[626.647762452972 24227.7055149319 24184.2785072302;376.991118430775 376.991118430775 376.991118430775;-0.546514462173508 0.180128407449521 1.73889282941709]  x3=[2.16604609549075 59.4665769231556 47.501237020576;376.991118430775 376.991118430775 376.991118430775;0.490744581019474 0.305731499154266 1.85850290347071]  x4=[1.88701911540475 82.2651467484152 70.3790856704584;376.991118430775 376.991118430775 376.991118430775;-1.97508293341556 0.0886602360035116 1.65757584201399]  x5=2.78556023988662e-06  V1=ones(3,3)  V2=ones(3,3)  I1=ones(3,3)  I2=ones(3,3)  nHarmo=1  Measurements=None
  836 : powerlib/Measurements/Three-Phase V-I Measurement  VoltageMeasurement=phase-to-ground  SetLabelV=on  LabelV=Vabc_836  Vpu=on  VpuLL=off  CurrentMeasurement=yes  SetLabelI=on  LabelI=Iabc_836  Ipu=on  Pbase=base_current  Vbase=Vnom_ph_ph  OutputType=Magnitude-Angle  PhasorSimulation=on  PSBequivalent=0
  836 D-I : powerlib/Elements/Three-Phase Series RLC Load  LConnTagsString=A|B|C  Configuration=Delta  NominalVoltage=[  Vabc=[1.017 1.025 1.02]*sqrt(3)*Vnom  Vabcp=V_836_840*Vnom  NominalFrequency=Frequency  UnbalancedPower=on  ActivePower=10e3  InductivePower=100  CapacitivePower=100  Pabc=[0 30 25]*1e3/2  QLabc=[0 15 14]*1e3/2  QCabc=[0 0 0]  Pabcp=Pa_836_840/2  QLabcp=Pp_836_840/2  QCabcp=Pn_836_840  Measurements=None  LoadType=constant I
      settings: AttributesFormatString=|
      | P= %<Pabc> W
      | Ql=%<QLabc> var
      | Qc=%<QCabc> var
  836 D-PQ : powerlib/Elements/Three-Phase Series RLC Load  LConnTagsString=A|B|C  Configuration=Delta  NominalVoltage=[  Vabc=[1.017 1.025 1.02]*sqrt(3)*Vnom  Vabcp=V_860_836*Vnom  NominalFrequency=Frequency  UnbalancedPower=on  ActivePower=10e3  InductivePower=100  CapacitivePower=100  Pabc=[0 30 25]*1e3/2  QLabc=[0 15 14]*1e3/2  QCabc=[0 0 0]  Pabcp=Pa_860_836/2  QLabcp=Pp_860_836/2  QCabcp=Pn_860_836  Measurements=None  LoadType=constant PQ
      settings: AttributesFormatString=|
      | P= %<Pabc> W
      | Ql=%<QLabc> var
      | Qc=%<QCabc> var
  836-840 : powerlib/Elements/Distributed Parameters Line  Phases=3  Frequency=Frequency  Resistance=R_301  Inductance=L_301  Capacitance=C_301  Length=860*ft2km  x1=[625.520414824784 24221.9054199327 24178.9038506397;376.991118430775 376.991118430775 376.991118430775;-0.541398558651721 0.180577064875552 1.73943786053142]  x2=[625.478839676754 24221.2670444385 24178.2138630858;376.991118430775 376.991118430775 376.991118430775;-0.541378322524158 0.180575906659205 1.73944570796266]  x3=[0.652627712821044 68.530359106575 57.0290618018578;376.991118430775 376.991118430775 376.991118430775;-0.434013331035901 0.191908795974235 1.76714643217602]  x4=[0.720170817088824 72.4484877514277 60.3507781317542;376.991118430775 376.991118430775 376.991118430775;-0.639085497603494 0.169502483650206 1.71291352791837]  x5=1.18593158727846e-06  V1=ones(3,3)  V2=ones(3,3)  I1=ones(3,3)  I2=ones(3,3)  nHarmo=1  Measurements=None
  836-862 : powerlib/Elements/Distributed Parameters Line  Phases=3  Frequency=Frequency  Resistance=R_301  Inductance=L_301  Capacitance=C_301  Length=280*ft2km  x1=[625.520499408163 24221.9052568694 24178.903806088;376.991118430775 376.991118430775 376.991118430775;-0.54109681672124 0.180822799537658 1.73967974948129]  x2=[625.439415435477 24221.779304539 24178.7945103371;376.991118430775 376.991118430775 376.991118430775;-0.540630025079495 0.180818192551836 1.7396841085015]  x3=[2.1087119712253 68.8822966096399 58.2510540944844;376.991118430775 376.991118430775 376.991118430775;0.197423003321293 0.173470328130528 1.76415042157582]  x4=[1.4324785009726 72.1499188882018 59.1612774186671;376.991118430775 376.991118430775 376.991118430775;-2.24736810769535 0.187721821526459 1.71547409013253]  x5=3.86117260974383e-07  V1=ones(3,3)  V2=ones(3,3)  I1=ones(3,3)  I2=ones(3,3)  nHarmo=1  Measurements=None
  838 : powerlib/Measurements/Three-Phase V-I Measurement  VoltageMeasurement=phase-to-ground  SetLabelV=on  LabelV=Vabc_838  Vpu=on  VpuLL=off  CurrentMeasurement=yes  SetLabelI=on  LabelI=Iabc_838  Ipu=on  Pbase=base_current  Vbase=Vnom_ph_ph  OutputType=Magnitude-Angle  PhasorSimulation=on  PSBequivalent=0
  838 Y-PQ : powerlib/Elements/Series RLC Load  LConnTagsString=a  RConnTagsString=__new0  NominalVoltage=V_862_838*Vnom  NominalFrequency=Frequency  ActivePower=Pa_862_838/2  InductivePower=Pp_862_838/2  CapacitivePower=Pn_862_838  Setx0=off  InitialVoltage=0  SetiL0=off  InitialCurrent=0  Measurements=None  LoadType=constant PQ
      settings: AttributesFormatString=|
      | P=%<ActivePower> W
      | Ql=%<InductivePower> var
      | Qc=%<CapacitivePower> var
  840 : powerlib/Measurements/Three-Phase V-I Measurement  VoltageMeasurement=phase-to-ground  SetLabelV=on  LabelV=Vabc_840  Vpu=on  VpuLL=off  CurrentMeasurement=yes  SetLabelI=on  LabelI=Iabc_840  Ipu=on  Pbase=base_current  Vbase=Vnom_ph_ph  OutputType=Magnitude-Angle  PhasorSimulation=on  PSBequivalent=0
  840 D-I : powerlib/Elements/Three-Phase Series RLC Load  LConnTagsString=A|B|C  Configuration=Delta  NominalVoltage=[  Vabc=[1.017 1.025 1.02]*sqrt(3)*Vnom  Vabcp=V_836_840*Vnom  NominalFrequency=Frequency  UnbalancedPower=on  ActivePower=10e3  InductivePower=100  CapacitivePower=100  Pabc=[0 30 25]*1e3/2  QLabc=[0 15 14]*1e3/2  QCabc=[0 0 0]  Pabcp=Pa_836_840/2  QLabcp=Pp_836_840/2  QCabcp=Pn_836_840  Measurements=None  LoadType=constant I
      settings: AttributesFormatString=|
      | P= %<Pabc> W
      | Ql=%<QLabc> var
      | Qc=%<QCabc> var
  840 Y-I : powerlib/Elements/Three-Phase Series RLC Load  LConnTagsString=A|B|C  Configuration=Y (grounded)  NominalVoltage=1000  Vabc=V_840*Vnom  Vabcp=[1e3 1e3 1e3]  NominalFrequency=Frequency  UnbalancedPower=on  ActivePower=10e3  InductivePower=100  CapacitivePower=100  Pabc=Pa_840  QLabc=Pp_840  QCabc=Pn_840  Pabcp=[10e3 9e3 11e3]  QLabcp=[100 90 110]  QCabcp=[100 90 110]  Measurements=None  LoadType=constant I
      settings: AttributesFormatString=|
      | P= %<Pabc> W
      | Ql=%<QLabc> var
      | Qc=%<QCabc> var
  842 : powerlib/Measurements/Three-Phase V-I Measurement  VoltageMeasurement=phase-to-ground  SetLabelV=on  LabelV=Vabc_842  Vpu=on  VpuLL=off  CurrentMeasurement=yes  SetLabelI=on  LabelI=Iabc_842  Ipu=on  Pbase=base_current  Vbase=Vnom_ph_ph  OutputType=Magnitude-Angle  PhasorSimulation=on  PSBequivalent=0
  842 Y-PQ : powerlib/Elements/Three-Phase Series RLC Load  LConnTagsString=A|B|C  Configuration=Y (grounded)  NominalVoltage=[  Vabc=V_842_844*Vnom  Vabcp=[1.031 1.029 1.031]*sqrt(3)*Vnom  NominalFrequency=Frequency  UnbalancedPower=on  ActivePower=10e3  InductivePower=100  CapacitivePower=100  Pabc=Pa_842_844/2  QLabc=Pp_842_844/2  QCabc=Pn_842_844  Pabcp=[16 20 110]*1e3/2  QLabcp=[8 10 55]*1e3/2  QCabcp=[0 0 0]  Measurements=None  LoadType=constant PQ
      settings: AttributesFormatString=|
      | P= %<Pabc> W
      | Ql=%<QLabc> var
      | Qc=%<QCabc> var
  842-844 : powerlib/Elements/Distributed Parameters Line  Phases=3  Frequency=Frequency  Resistance=R_301  Inductance=L_301  Capacitance=C_301  Length=1350*ft2km  x1=[628.151716180336 24237.5914731138 24194.2083063583;376.991118430775 376.991118430775 376.991118430775;-0.549650005196056 0.180127426608067 1.73896664934359]  x2=[628.688384281081 24239.0234928775 24196.9130558911;376.991118430775 376.991118430775 376.991118430775;-0.550336547844137 0.179044647602196 1.73791226985305]  x3=[1.0783502023434 72.0707805960007 62.1394657567476;376.991118430775 376.991118430775 376.991118430775;-1.36428160290148 -0.617310357777565 0.840914426345981]  x4=[1.0065419296097 104.256733421505 92.416878424627;376.991118430775 376.991118430775 376.991118430775;0.342503839618023 0.696283098022532 2.29150868076604]  x5=1.86163679398363e-06  V1=ones(3,3)  V2=ones(3,3)  I1=ones(3,3)  I2=ones(3,3)  nHarmo=1  Measurements=None
  844 : powerlib/Measurements/Three-Phase V-I Measurement  VoltageMeasurement=phase-to-ground  SetLabelV=on  LabelV=Vabc_844  Vpu=on  VpuLL=off  CurrentMeasurement=yes  SetLabelI=on  LabelI=Iabc_844  Ipu=on  Pbase=base_current  Vbase=Vnom_ph_ph  OutputType=Magnitude-Angle  PhasorSimulation=on  PSBequivalent=0
  844 Y-PQ : powerlib/Elements/Three-Phase Series RLC Load  LConnTagsString=A|B|C  Configuration=Y (grounded)  NominalVoltage=[  Vabc=V_842_844*Vnom  Vabcp=[1.031 1.029 1.031]*sqrt(3)*Vnom  NominalFrequency=Frequency  UnbalancedPower=on  ActivePower=10e3  InductivePower=100  CapacitivePower=100  Pabc=Pa_842_844/2  QLabc=Pp_842_844/2  QCabc=Pn_842_844  Pabcp=[16 20 110]*1e3/2  QLabcp=[8 10 55]*1e3/2  QCabcp=[0 0 0]  Measurements=None  LoadType=constant PQ
      settings: AttributesFormatString=|
      | P= %<Pabc> W
      | Ql=%<QLabc> var
      | Qc=%<QCabc> var
  844 Y-PQ1 : powerlib/Elements/Three-Phase Series RLC Load  LConnTagsString=A|B|C  Configuration=Y (grounded)  NominalVoltage=[  Vabc=V_844_846*Vnom  Vabcp=[1.031 1.029 1.031]*sqrt(3)*Vnom  NominalFrequency=Frequency  UnbalancedPower=on  ActivePower=10e3  InductivePower=100  CapacitivePower=100  Pabc=Pa_844_846/2  QLabc=Pp_844_846/2  QCabc=Pn_844_846  Pabcp=[16 20 110]*1e3/2  QLabcp=[8 10 55]*1e3/2  QCabcp=[0 0 0]  Measurements=None  LoadType=constant PQ
      settings: AttributesFormatString=|
      | P= %<Pabc> W
      | Ql=%<QLabc> var
      | Qc=%<QCabc> var
  844 Y-Z : powerlib/Elements/Three-Phase Series RLC Load  LConnTagsString=A|B|C  Configuration=Y (grounded)  NominalVoltage=[  Vabc=V_844*Vnom  Vabcp=[1.031 1.029 1.031]*sqrt(3)*Vnom  NominalFrequency=Frequency  UnbalancedPower=on  ActivePower=10e3  InductivePower=100  CapacitivePower=100  Pabc=Pa_844  QLabc=Pp_844  QCabc=[0 0 0]  Pabcp=[16 20 110]*1e3/2  QLabcp=[8 10 55]*1e3/2  QCabcp=[0 0 0]  Measurements=Branch voltages and currents  LoadType=constant Z
      settings: AttributesFormatString=|
      | P= %<Pabc> W
      | Ql=%<QLabc> var
      | Qc=%<QCabc> var
  844 Y-Z1 : powerlib/Elements/Three-Phase Series RLC Load  LConnTagsString=A|B|C  Configuration=Y (grounded)  NominalVoltage=[  Vabc="[1  1  1]*Vnom"  Vabcp=[1.031 1.029 1.031]*sqrt(3)*Vnom  NominalFrequency=Frequency  UnbalancedPower=on  ActivePower=10e3  InductivePower=100  CapacitivePower=100  Pabc=[0 0 0]  QLabc=[0 0 0]  QCabc=Pn_844  Pabcp=[16 20 110]*1e3/2  QLabcp=[8 10 55]*1e3/2  QCabcp=[0 0 0]  Measurements=None  LoadType=constant Z
      settings: AttributesFormatString=|
      | P= %<Pabc> W
      | Ql=%<QLabc> var
      | Qc=%<QCabc> var
  844-846 : powerlib/Elements/Distributed Parameters Line  Phases=3  Frequency=Frequency  Resistance=R_301  Inductance=L_301  Capacitance=C_301  Length=3640*ft2km  x1=[628.688384281081 24239.0234928776 24196.9130558911;376.991118430775 376.991118430775 376.991118430775;-0.551527043421843 0.178074411129144 1.73695724832462]  x2=[630.84660081719 24261.4645339968 24223.3419894264;376.991118430775 376.991118430775 376.991118430775;-0.553739359109096 0.175505407445902 1.73450065798007]  x3=[1.38154681988528 83.8611516362285 73.6675492850921;376.991118430775 376.991118430775 376.991118430775;-1.43930769245329 -0.483869338145208 1.00430494604313]  x4=[1.18065623220157 90.6044595685841 79.4704147154107;376.991118430775 376.991118430775 376.991118430775;0.580475245644143 0.77936545449448 2.40197129158137]  x5=5.01952439266698e-06  V1=ones(3,3)  V2=ones(3,3)  I1=ones(3,3)  I2=ones(3,3)  nHarmo=1  Measurements=None
  846 : powerlib/Measurements/Three-Phase V-I Measurement  VoltageMeasurement=phase-to-ground  SetLabelV=on  LabelV=Vabc_846  Vpu=on  VpuLL=off  CurrentMeasurement=yes  SetLabelI=on  LabelI=Iabc_846  Ipu=on  Pbase=base_current  Vbase=Vnom_ph_ph  OutputType=Magnitude-Angle  PhasorSimulation=on  PSBequivalent=0
  846 Y-PQ : powerlib/Elements/Three-Phase Series RLC Load  LConnTagsString=A|B|C  Configuration=Y (grounded)  NominalVoltage=[  Vabc=V_844_846*Vnom  Vabcp=[1.031 1.029 1.031]*sqrt(3)*Vnom  NominalFrequency=Frequency  UnbalancedPower=on  ActivePower=10e3  InductivePower=100  CapacitivePower=100  Pabc=Pa_844_846/2  QLabc=Pp_844_846/2  QCabc=Pn_844_846  Pabcp=[16 20 110]*1e3/2  QLabcp=[8 10 55]*1e3/2  QCabcp=[0 0 0]  Measurements=None  LoadType=constant PQ
      settings: AttributesFormatString=|
      | P= %<Pabc> W
      | Ql=%<QLabc> var
      | Qc=%<QCabc> var
  846 Y-PQ1 : powerlib/Elements/Three-Phase Series RLC Load  LConnTagsString=A|B|C  Configuration=Y (grounded)  NominalVoltage=[  Vabc=V_846_848*Vnom  Vabcp=[1.031 1.029 1.031]*sqrt(3)*Vnom  NominalFrequency=Frequency  UnbalancedPower=on  ActivePower=10e3  InductivePower=100  CapacitivePower=100  Pabc=Pa_846_848/2  QLabc=Pp_846_848/2  QCabc=Pn_846_848  Pabcp=[16 20 110]*1e3/2  QLabcp=[8 10 55]*1e3/2  QCabcp=[0 0 0]  Measurements=None  LoadType=constant PQ
      settings: AttributesFormatString=|
      | P= %<Pabc> W
      | Ql=%<QLabc> var
      | Qc=%<QCabc> var
  846-848 : powerlib/Elements/Distributed Parameters Line  Phases=3  Frequency=Frequency  Resistance=R_301  Inductance=L_301  Capacitance=C_301  Length=530*ft2km  x1=[630.84660081719 24261.4645339968 24223.3419894264;376.991118430775 376.991118430775 376.991118430775;-0.552122572538498 0.176823064839435 1.73579765228288]  x2=[631.108008491299 24264.9529214849 24227.5344376335;376.991118430775 376.991118430775 376.991118430775;-0.553104820101629 0.176455720788207 1.7354350271986]  x3=[1.78598057926325 85.0579658643375 75.7447500458602;376.991118430775 376.991118430775 376.991118430775;-2.18953088248425 -0.470538278445313 1.00202072147218]  x4=[2.32644410942973 89.5213227281586 79.5705668754173;376.991118430775 376.991118430775 376.991118430775;0.319869286339696 0.786433560051124 2.4264618855554]  x5=7.30864815415796e-07  V1=ones(3,3)  V2=ones(3,3)  I1=ones(3,3)  I2=ones(3,3)  nHarmo=1  Measurements=None
  848 : powerlib/Measurements/Three-Phase V-I Measurement  VoltageMeasurement=phase-to-ground  SetLabelV=on  LabelV=Vabc_848  Vpu=on  VpuLL=off  CurrentMeasurement=yes  SetLabelI=on  LabelI=Iabc_848  Ipu=on  Pbase=base_current  Vbase=Vnom_ph_ph  OutputType=Magnitude-Angle  PhasorSimulation=on  PSBequivalent=0
  848 D-PQ : powerlib/Elements/Three-Phase Series RLC Load  LConnTagsString=A|B|C  Configuration=Delta  NominalVoltage=1000  Vabc=[1e3 1e3 1e3]  Vabcp=V_848*Vnom  NominalFrequency=Frequency  UnbalancedPower=on  ActivePower=[20 20 20]*1e3  InductivePower=[20 20 20]*1e3  CapacitivePower=100  Pabc=[10e3 9e3 11e3]  QLabc=[100 90 110]  QCabc=[100 90 110]  Pabcp=Pa_848  QLabcp=Pp_848  QCabcp=[0 0 0]  Measurements=Branch voltages and currents  LoadType=constant PQ
      settings: AttributesFormatString=|
      | P= %<Pabc> W
      | Ql=%<QLabc> var
      | Qc=%<QCabc> var
  848 D-Z : powerlib/Elements/Three-Phase Series RLC Load  LConnTagsString=A|B|C  Configuration=Delta  NominalVoltage=1000  Vabc=[1e3 1e3 1e3]  Vabcp="[1  1  1]*Vnom"  NominalFrequency=Frequency  UnbalancedPower=on  ActivePower=[20 20 20]*1e3  InductivePower=[20 20 20]*1e3  CapacitivePower=100  Pabc=[10e3 9e3 11e3]  QLabc=[100 90 110]  QCabc=[100 90 110]  Pabcp=[0 0 0]  QLabcp=[0 0 0]  QCabcp=Pn_848  Measurements=None  LoadType=constant Z
      settings: AttributesFormatString=|
      | P= %<Pabc> W
      | Ql=%<QLabc> var
      | Qc=%<QCabc> var
  848 Y-PQ : powerlib/Elements/Three-Phase Series RLC Load  LConnTagsString=A|B|C  Configuration=Y (grounded)  NominalVoltage=[  Vabc=V_846_848*Vnom  Vabcp=[1.031 1.029 1.031]*sqrt(3)*Vnom  NominalFrequency=Frequency  UnbalancedPower=on  ActivePower=10e3  InductivePower=100  CapacitivePower=100  Pabc=Pa_846_848/2  QLabc=Pp_846_848/2  QCabc=Pn_846_848  Pabcp=[16 20 110]*1e3/2  QLabcp=[8 10 55]*1e3/2  QCabcp=[0 0 0]  Measurements=None  LoadType=constant PQ
      settings: AttributesFormatString=|
      | P= %<Pabc> W
      | Ql=%<QLabc> var
      | Qc=%<QCabc> var
  850 : powerlib/Measurements/Three-Phase V-I Measurement  VoltageMeasurement=phase-to-ground  SetLabelV=on  LabelV=Vabc_850  Vpu=on  VpuLL=off  CurrentMeasurement=yes  SetLabelI=on  LabelI=Iabc_850  Ipu=on  Pbase=base_current  Vbase=Vnom_ph_ph  OutputType=Magnitude-Angle  PhasorSimulation=on  PSBequivalent=0
  850-816 : powerlib/Elements/Distributed Parameters Line  Phases=3  Frequency=Frequency  Resistance=R_301  Inductance=L_301  Capacitance=C_301  Length=310*ft2km  x1=[749.130109468562 25226.871106407 25140.5627784305;376.991118430775 376.991118430775 376.991118430775;-0.624201015313123 0.237482476073869 1.80401481502904]  x2=[748.410739748618 25222.2511977151 25136.0453810114;376.991118430775 376.991118430775 376.991118430775;-0.623475804516978 0.237262794077505 1.80377524400646]  x3=[4.47466479164296 31.8766496158322 28.1236135299063;376.991118430775 376.991118430775 376.991118430775;0.864096343342865 -0.885650882773149 0.234602118570318]  x4=[4.63531202065509 136.127568250359 125.18892988738;376.991118430775 376.991118430775 376.991118430775;-1.91828966649123 0.449981676961245 2.0304132999877]  x5=4.27486967507352e-07  V1=ones(3,3)  V2=ones(3,3)  I1=ones(3,3)  I2=ones(3,3)  nHarmo=1  Measurements=None
  852 : powerlib/Measurements/Three-Phase V-I Measurement  VoltageMeasurement=phase-to-ground  SetLabelV=on  LabelV=Vabc_852  Vpu=on  VpuLL=off  CurrentMeasurement=yes  SetLabelI=on  LabelI=Iabc_852  Ipu=on  Pbase=base_current  Vbase=Vnom_ph_ph  OutputType=Magnitude-Angle  PhasorSimulation=on  PSBequivalent=0
  852-832 : powerlib/Elements/Distributed Parameters Line  Phases=3  Frequency=Frequency  Resistance=R_301  Inductance=L_301  Capacitance=C_301  Length=10*ft2km  x1=[635.235940245995 24292.5908336149 24240.4839975325;376.991118430775 376.991118430775 376.991118430775;-0.557646726157538 0.188875409186031 1.74857049690205]  x2=[635.221909871997 24292.4633816385 24240.3627284127;376.991118430775 376.991118430775 376.991118430775;-0.557638251549899 0.188868244306889 1.74856231182074]  x3=[2.15773077380983 34.6518416216895 32.5147245428087;376.991118430775 376.991118430775 376.991118430775;1.09028158247579 -0.861535269014886 0.278441295595743]  x4=[2.65360636603915 127.82330780218 118.912057175277;376.991118430775 376.991118430775 376.991118430775;-1.50301567338363 0.426300083014506 2.02408765803074]  x5=1.37899021776565e-08  V1=ones(3,3)  V2=ones(3,3)  I1=ones(3,3)  I2=ones(3,3)  nHarmo=1  Measurements=None
  854 : powerlib/Measurements/Three-Phase V-I Measurement  VoltageMeasurement=phase-to-ground  SetLabelV=on  LabelV=Vabc_854  Vpu=on  VpuLL=off  CurrentMeasurement=yes  SetLabelI=on  LabelI=Iabc_854  Ipu=on  Pbase=base_current  Vbase=Vnom_ph_ph  OutputType=Magnitude-Angle  PhasorSimulation=on  PSBequivalent=0
  854 Y-PQ : powerlib/Elements/Series RLC Load  LConnTagsString=a  RConnTagsString=__new0  NominalVoltage=V_854_856*Vnom  NominalFrequency=Frequency  ActivePower=Pa_854_856/2  InductivePower=Pp_854_856/2  CapacitivePower=Pn_854_856  Setx0=off  InitialVoltage=0  SetiL0=off  InitialCurrent=0  Measurements=None  LoadType=constant PQ
      settings: AttributesFormatString=|
      | P=%<ActivePower> W
      | Ql=%<InductivePower> var
      | Qc=%<CapacitivePower> var
  854-852 : powerlib/Elements/Distributed Parameters Line  Phases=3  Frequency=Frequency  Resistance=R_301  Inductance=L_301  Capacitance=C_301  Length=36830*ft2km  x1=[687.074296441229 24767.4205301758 24695.151726903;376.991118430775 376.991118430775 376.991118430775;-0.60548484623889 0.199423981829368 1.76302473691249]  x2=[635.235940245995 24292.5908336149 24240.4839975325;376.991118430775 376.991118430775 376.991118430775;-0.576788231472449 0.173275362488311 1.73321508525274]  x3=[2.10041992160321 33.80505197171 31.2849315274215;376.991118430775 376.991118430775 376.991118430775;1.04758558606382 -0.84705016997366 0.286754445921044]  x4=[2.62844707464827 125.075465727344 116.839399182622;376.991118430775 376.991118430775 376.991118430775;-1.52308776962872 0.411817303931343 2.00969116370023]  x5=5.0788209720309e-05  V1=ones(3,3)  V2=ones(3,3)  I1=ones(3,3)  I2=ones(3,3)  nHarmo=1  Measurements=None
  854-856 : powerlib/Elements/Distributed Parameters Line  Phases=1  Frequency=Frequency  Resistance=R_303(2,2)  Inductance=L_303(2,2)  Capacitance=C_303(2,2)  Length=23330*ft2km  x1=[20198.6382796467;376.991118430775;-2.20056250783936]  x2=[20196.8042831139;376.991118430775;-2.20068164791828]  x3=[33.3432195456352;376.991118430775;-2.20884130198352]  x4=[33.7275884775758;376.991118430775;-2.20356056658947]  x5=2.9363349960162e-05  V1=ones(3,3)  V2=ones(3,3)  I1=ones(3,3)  I2=ones(3,3)  nHarmo=1  Measurements=None
  856 : powerlib/Measurements/Three-Phase V-I Measurement  VoltageMeasurement=phase-to-ground  SetLabelV=on  LabelV=Vabc_856  Vpu=on  VpuLL=off  CurrentMeasurement=yes  SetLabelI=on  LabelI=Iabc_856  Ipu=on  Pbase=base_current  Vbase=Vnom_ph_ph  OutputType=Magnitude-Angle  PhasorSimulation=on  PSBequivalent=0
  856 Y-PQ : powerlib/Elements/Series RLC Load  LConnTagsString=a  RConnTagsString=__new0  NominalVoltage=V_854_856*Vnom  NominalFrequency=Frequency  ActivePower=Pa_854_856/2  InductivePower=Pp_854_856/2  CapacitivePower=Pn_854_856  Setx0=off  InitialVoltage=0  SetiL0=off  InitialCurrent=0  Measurements=None  LoadType=constant PQ
      settings: AttributesFormatString=|
      | P=%<ActivePower> W
      | Ql=%<InductivePower> var
      | Qc=%<CapacitivePower> var
  858 : powerlib/Measurements/Three-Phase V-I Measurement  VoltageMeasurement=phase-to-ground  SetLabelV=on  LabelV=Vabc_858  Vpu=on  VpuLL=off  CurrentMeasurement=yes  SetLabelI=on  LabelI=Iabc_858  Ipu=on  Pbase=base_current  Vbase=Vnom_ph_ph  OutputType=Magnitude-Angle  PhasorSimulation=on  PSBequivalent=0
  858 D-PQ : powerlib/Elements/Three-Phase Series RLC Load  LConnTagsString=A|B|C  Configuration=Delta  NominalVoltage=[  Vabc=[1.017 1.025 1.02]*sqrt(3)*Vnom  Vabcp=V_858_834*Vnom  NominalFrequency=Frequency  UnbalancedPower=on  ActivePower=10e3  InductivePower=100  CapacitivePower=100  Pabc=[0 30 25]*1e3/2  QLabc=[0 15 14]*1e3/2  QCabc=[0 0 0]  Pabcp=Pa_858_834/2  QLabcp=Pp_858_834/2  QCabcp=Pn_858_834  Measurements=None  LoadType=constant PQ
      settings: AttributesFormatString=|
      | P= %<Pabc> W
      | Ql=%<QLabc> var
      | Qc=%<QCabc> var
  858 D-Z : powerlib/Elements/Three-Phase Series RLC Load  LConnTagsString=A|B|C  Configuration=Delta  NominalVoltage=[  Vabc=[1.017 1.025 1.02]*sqrt(3)*Vnom  Vabcp=V_832_858*Vnom  NominalFrequency=Frequency  UnbalancedPower=on  ActivePower=10e3  InductivePower=100  CapacitivePower=100  Pabc=[0 30 25]*1e3/2  QLabc=[0 15 14]*1e3/2  QCabc=[0 0 0]  Pabcp=Pa_832_858/2  QLabcp=Pp_832_858/2  QCabcp=Pn_832_858  Measurements=None  LoadType=constant Z
      settings: AttributesFormatString=|
      | P= %<Pabc> W
      | Ql=%<QLabc> var
      | Qc=%<QCabc> var
  858 Y-PQ : powerlib/Elements/Series RLC Load  LConnTagsString=a  RConnTagsString=__new0  NominalVoltage=1.034*Vnom  NominalFrequency=Frequency  ActivePower=Pa_858_864/2  InductivePower=Pp_858_864/2  CapacitivePower=Pn_858_864  Setx0=off  InitialVoltage=0  SetiL0=off  InitialCurrent=0  Measurements=None  LoadType=constant PQ
      settings: AttributesFormatString=|
      | P=%<ActivePower> W
      | Ql=%<InductivePower> var
      | Qc=%<CapacitivePower> var
  858-834 : powerlib/Elements/Distributed Parameters Line  Phases=3  Frequency=Frequency  Resistance=R_301  Inductance=L_301  Capacitance=C_301  Length=5830*ft2km  x1=[631.73772567187 24266.2453880144 24217.7971104675;376.991118430775 376.991118430775 376.991118430775;-0.556874781291206 0.182776975148309 1.74210218697933]  x2=[628.077484124564 24237.3315138492 24193.654603702;376.991118430775 376.991118430775 376.991118430775;-0.551780220586984 0.178453700837703 1.73731770402779]  x3=[1.43931904997291 54.5226268037395 48.295880625088;376.991118430775 376.991118430775 376.991118430775;0.544849674942409 -0.658216499035748 0.653502951647773]  x4=[1.47177338120119 111.767715694311 103.77576820456;376.991118430775 376.991118430775 376.991118430775;-1.61485093796653 0.550295391289653 2.16263864539096]  x5=8.03951296957376e-06  V1=ones(3,3)  V2=ones(3,3)  I1=ones(3,3)  I2=ones(3,3)  nHarmo=1  Measurements=None
  858-864 : powerlib/Elements/Distributed Parameters Line  Phases=1  Frequency=Frequency  Resistance=R_302(1,1)  Inductance=L_302(1,1)  Capacitance=C_302(1,1)  Length=1620*ft2km  x1=[19656.4785913675;376.991118430775;-0.102695438129856]  x2=[19656.3877161081;376.991118430775;-0.102696113935644]  x3=[33.0254499715375;376.991118430775;-0.102120612056694]  x4=[33.2031084111784;376.991118430775;-0.104034748498426]  x5=2.03894671819385e-06  V1=ones(3,3)  V2=ones(3,3)  I1=ones(3,3)  I2=ones(3,3)  nHarmo=1  Measurements=None
  860 : powerlib/Measurements/Three-Phase V-I Measurement  VoltageMeasurement=phase-to-ground  SetLabelV=on  LabelV=Vabc_860  Vpu=on  VpuLL=off  CurrentMeasurement=yes  SetLabelI=on  LabelI=Iabc_860  Ipu=on  Pbase=base_current  Vbase=Vnom_ph_ph  OutputType=Magnitude-Angle  PhasorSimulation=on  PSBequivalent=0
  860 D-PQ : powerlib/Elements/Three-Phase Series RLC Load  LConnTagsString=A|B|C  Configuration=Delta  NominalVoltage=[  Vabc=[1.017 1.025 1.02]*sqrt(3)*Vnom  Vabcp=V_860_836*Vnom  NominalFrequency=Frequency  UnbalancedPower=on  ActivePower=10e3  InductivePower=100  CapacitivePower=100  Pabc=[0 30 25]*1e3/2  QLabc=[0 15 14]*1e3/2  QCabc=[0 0 0]  Pabcp=Pa_860_836/2  QLabcp=Pp_860_836/2  QCabcp=Pn_860_836  Measurements=None  LoadType=constant PQ
      settings: AttributesFormatString=|
      | P= %<Pabc> W
      | Ql=%<QLabc> var
      | Qc=%<QCabc> var
  860 D-Z : powerlib/Elements/Three-Phase Series RLC Load  LConnTagsString=A|B|C  Configuration=Delta  NominalVoltage=[  Vabc=[1.017 1.025 1.02]*sqrt(3)*Vnom  Vabcp=V_834_860*Vnom  NominalFrequency=Frequency  UnbalancedPower=on  ActivePower=10e3  InductivePower=100  CapacitivePower=100  Pabc=[0 30 25]*1e3/2  QLabc=[0 15 14]*1e3/2  QCabc=[0 0 0]  Pabcp=Pa_834_860/2  QLabcp=Pp_834_860/2  QCabcp=Pn_834_860  Measurements=None  LoadType=constant Z
      settings: AttributesFormatString=|
      | P= %<Pabc> W
      | Ql=%<QLabc> var
      | Qc=%<QCabc> var
  860 Y-PQ : powerlib/Elements/Three-Phase Series RLC Load  LConnTagsString=A|B|C  Configuration=Y (grounded)  NominalVoltage=[  Vabc=V_860*Vnom  Vabcp=[1.031 1.029 1.031]*sqrt(3)*Vnom  NominalFrequency=Frequency  UnbalancedPower=on  ActivePower=10e3  InductivePower=100  CapacitivePower=100  Pabc=Pa_860  QLabc=Pp_860  QCabc=Pn_860  Pabcp=[16 20 110]*1e3/2  QLabcp=[8 10 55]*1e3/2  QCabcp=[0 0 0]  Measurements=None  LoadType=constant PQ
      settings: AttributesFormatString=|
      | P= %<Pabc> W
      | Ql=%<QLabc> var
      | Qc=%<QCabc> var
  860-836 : powerlib/Elements/Distributed Parameters Line  Phases=3  Frequency=Frequency  Resistance=R_301  Inductance=L_301  Capacitance=C_301  Length=2680*ft2km  x1=[626.647762452972 24227.7055149319 24184.2785072302;376.991118430775 376.991118430775 376.991118430775;-0.546857574436079 0.179848775976938 1.73861758303772]  x2=[625.520414824784 24221.9054199327 24178.9038506397;376.991118430775 376.991118430775 376.991118430775;-0.542344716709112 0.179805959905703 1.7386788477883]  x3=[2.13250437810903 64.3779057300328 54.6130472959515;376.991118430775 376.991118430775 376.991118430775;0.287629430685251 0.203223592681619 1.81088250189155]  x4=[1.57934071523055 76.4657409617383 62.8849498556472;376.991118430775 376.991118430775 376.991118430775;-2.15953190341272 0.159083848320397 1.67488468396614]  x5=3.69569378361195e-06  V1=ones(3,3)  V2=ones(3,3)  I1=ones(3,3)  I2=ones(3,3)  nHarmo=1  Measurements=None
  862 : powerlib/Measurements/Three-Phase V-I Measurement  VoltageMeasurement=phase-to-ground  SetLabelV=on  LabelV=Vabc_862  Vpu=on  VpuLL=off  CurrentMeasurement=yes  SetLabelI=on  LabelI=Iabc_862  Ipu=on  Pbase=base_current  Vbase=Vnom_ph_ph  OutputType=Magnitude-Angle  PhasorSimulation=on  PSBequivalent=0
  862 Y-PQ : powerlib/Elements/Series RLC Load  LConnTagsString=a  RConnTagsString=__new0  NominalVoltage=V_862_838*Vnom  NominalFrequency=Frequency  ActivePower=Pa_862_838/2  InductivePower=Pp_862_838/2  CapacitivePower=Pn_862_838  Setx0=off  InitialVoltage=0  SetiL0=off  InitialCurrent=0  Measurements=None  LoadType=constant PQ
      settings: AttributesFormatString=|
      | P=%<ActivePower> W
      | Ql=%<InductivePower> var
      | Qc=%<CapacitivePower> var
  862-838 : powerlib/Elements/Distributed Parameters Line  Phases=1  Frequency=Frequency  Resistance=R_304(2,2)  Inductance=L_304(2,2)  Capacitance=C_304(2,2)  Length=4860*ft2km  x1=[19777.8290488467;376.991118430775;-2.22884089285595]  x2=[19774.8157081551;376.991118430775;-2.22887154960352]  x3=[33.3169781587749;376.991118430775;-2.21226271609078]  x4=[35.8390045864165;376.991118430775;-2.24649519699912]  x5=6.08033278760362e-06  V1=ones(3,3)  V2=ones(3,3)  I1=ones(3,3)  I2=ones(3,3)  nHarmo=1  Measurements=None
  864 : powerlib/Measurements/Three-Phase V-I Measurement  VoltageMeasurement=phase-to-ground  SetLabelV=on  LabelV=Vabc_864  Vpu=on  VpuLL=off  CurrentMeasurement=yes  SetLabelI=on  LabelI=Iabc_864  Ipu=on  Pbase=base_current  Vbase=Vnom_ph_ph  OutputType=Magnitude-Angle  PhasorSimulation=on  PSBequivalent=0
  864 Y-PQ : powerlib/Elements/Series RLC Load  LConnTagsString=a  RConnTagsString=__new0  NominalVoltage=1.034*Vnom  NominalFrequency=Frequency  ActivePower=2e3/2  InductivePower=1e3/2  CapacitivePower=0  Setx0=off  InitialVoltage=0  SetiL0=off  InitialCurrent=0  Measurements=None  LoadType=constant PQ
      settings: AttributesFormatString=|
      | P=%<ActivePower> W
      | Ql=%<InductivePower> var
      | Qc=%<CapacitivePower> var
  888 : powerlib/Measurements/Three-Phase V-I Measurement  VoltageMeasurement=phase-to-ground  SetLabelV=on  LabelV=Vabc_888  Vpu=on  VpuLL=off  CurrentMeasurement=yes  SetLabelI=on  LabelI=Iabc_888  Ipu=on  Pbase=base_current  Vbase=Vnom1_ph_ph  OutputType=Magnitude-Angle  PhasorSimulation=on  PSBequivalent=0
  888-890 : powerlib/Elements/Distributed Parameters Line  Phases=3  Frequency=Frequency  Resistance=R_300  Inductance=L_300  Capacitance=C_300  Length=10560*ft2km  x1=[255.288690360266 3904.11861787347 3893.29669211033;376.991118430775 376.991118430775 376.991118430775;1.80415691993535 0.156851370671844 1.71914594840713]  x2=[268.985758469987 3572.87147233613 3550.21045154299;376.991118430775 376.991118430775 376.991118430775;1.86910597942955 0.145360509232767 1.69994914932308]  x3=[4.27995630496126 112.784264651167 114.043119709179;376.991118430775 376.991118430775 376.991118430775;1.79651787069956 2.77832077505203 -1.94512698637707]  x4=[3.64804604698998 132.658110647829 130.464904862869;376.991118430775 376.991118430775 376.991118430775;-1.35171120472639 -0.280826828764399 1.26579376866958]  x5=1.41710191462344e-05  V1=ones(3,3)  V2=ones(3,3)  I1=ones(3,3)  I2=ones(3,3)  nHarmo=1  Measurements=None
  890 : powerlib/Measurements/Three-Phase V-I Measurement  VoltageMeasurement=phase-to-ground  SetLabelV=on  LabelV=Vabc_890  Vpu=on  VpuLL=off  CurrentMeasurement=yes  SetLabelI=on  LabelI=Iabc_890  Ipu=on  Pbase=base_current  Vbase=Vnom1_ph_ph  OutputType=Magnitude-Angle  PhasorSimulation=on  PSBequivalent=0
  890 D-I : powerlib/Elements/Three-Phase Series RLC Load  LConnTagsString=A|B|C  Configuration=Delta  NominalVoltage=1000  Vabc=[1e3 1e3 1e3]  Vabcp=V_890*Vnom1  NominalFrequency=Frequency  UnbalancedPower=on  ActivePower=10e3  InductivePower=100  CapacitivePower=100  Pabc=[10e3 9e3 11e3]  QLabc=[100 90 110]  QCabc=[100 90 110]  Pabcp=Pa_890  QLabcp=Pp_890  QCabcp=Pn_890  Measurements=None  LoadType=constant I
  Breaker818-820 : powerlib/Elements/Breaker  InitialState=0  SwitchingTimes="[1/60  5/60]"  External=on  BreakerResistance=0.0001  SnubberResistance=inf  SnubberCapacitance=0  Measurements=None  MoreParameters=on  NoBreakLoop=off
  Breaker832-858 : powerlib/Elements/Three-Phase Breaker  InitialState=closed  SwitchA=on  SwitchB=on  SwitchC=on  SwitchTimes=[0.5 ]  External=on  BreakerResistance=0.0001  SnubberResistance=inf  SnubberCapacitance=0  Measurements=None
  Breaker834-842 : powerlib/Elements/Three-Phase Breaker  InitialState=closed  SwitchA=on  SwitchB=on  SwitchC=on  SwitchTimes=[0.5 ]  External=on  BreakerResistance=0.0001  SnubberResistance=inf  SnubberCapacitance=0  Measurements=None
  Breaker836-862 : powerlib/Elements/Three-Phase Breaker  InitialState=closed  SwitchA=on  SwitchB=on  SwitchC=on  SwitchTimes=[0.5 ]  External=on  BreakerResistance=0.0001  SnubberResistance=inf  SnubberCapacitance=0  Measurements=None
  Breaker850-816 : powerlib/Elements/Three-Phase Breaker  InitialState=closed  SwitchA=on  SwitchB=on  SwitchC=on  SwitchTimes=[0.5 ]  External=on  BreakerResistance=0.0001  SnubberResistance=inf  SnubberCapacitance=0  Measurements=None
  Constant1 : Constant  Value=SW850_816
  Constant2 : Constant  Value=SW818_820
  Constant3 : Constant  Value=SW832_858
  Constant4 : Constant  Value=SW834_842
  Constant5 : Constant  Value=SW836_862
  Ground{,1..21} (22 alike) : powerlib/Elements/Ground  LConnTagsString=a
  Load Flow Bus : powerlib/Measurements/Load Flow Bus  LConnTagsString=a|b|c  RConnTagsString=a|b|c  Phases=ABC  Connectors=on both sides  ID=800  Vbase=Vnom  Vref="[1.05  1.05  1.05]"  Vangle="[0  -120  120]"  VLF=1  VLFb=1  VLFc=1  angleLF=0  angleLFb=0  angleLFc=0
      settings: AttributesFormatString=%<ID>
  Load Flow Bus1 : powerlib/Measurements/Load Flow Bus  LConnTagsString=a|b|c  RConnTagsString=a|b|c  Phases=ABC  Connectors=on both sides  ID=802  Vbase=Vnom  Vref=[1.0475 1.0484 1.0484]  Vangle=[-0.05 -120.07 119.95]  VLF=1  VLFb=1  VLFc=1  angleLF=0  angleLFb=0  angleLFc=0
      settings: AttributesFormatString=%<ID>
  Load Flow Bus10 : powerlib/Measurements/Load Flow Bus  LConnTagsString=a  Phases=B  Connectors=on one side  ID=826  Vbase=Vnom  Vref=1.0156  Vangle=-122.94  VLF=1  VLFb=1  VLFc=1  angleLF=0  angleLFb=0  angleLFc=0
      settings: AttributesFormatString=%<ID>
  Load Flow Bus11 : powerlib/Measurements/Load Flow Bus  LConnTagsString=a  RConnTagsString=a  Phases=A  Connectors=on both sides  ID=818  Vbase=Vnom  Vref=1.0163  Vangle=-2.27  VLF=1  VLFb=1  VLFc=1  angleLF=0  angleLFb=0  angleLFc=0
      settings: AttributesFormatString=%<ID>
  Load Flow Bus12 : powerlib/Measurements/Load Flow Bus  LConnTagsString=a  RConnTagsString=a  Phases=A  Connectors=on both sides  ID=820  Vbase=Vnom  Vref=0.9926  Vangle=-2.32  VLF=1  VLFb=1  VLFc=1  angleLF=0  angleLFb=0  angleLFc=0
      settings: AttributesFormatString=%<ID>
  Load Flow Bus13 : powerlib/Measurements/Load Flow Bus  LConnTagsString=a  Phases=A  Connectors=on one side  ID=822  Vbase=Vnom  Vref=0.9895  Vangle=-2.33  VLF=1  VLFb=1  VLFc=1  angleLF=0  angleLFb=0  angleLFc=0
      settings: AttributesFormatString=%<ID>
  Load Flow Bus14 : powerlib/Measurements/Load Flow Bus  LConnTagsString=a|b|c  RConnTagsString=a|b|c  Phases=ABC  Connectors=on both sides  ID=828  Vbase=Vnom  Vref=[1.0074 1.0151 1.0109]  Vangle=[-2.38 -122.95 117.75]  VLF=1  VLFb=1  VLFc=1  angleLF=0  angleLFb=0  angleLFc=0
      settings: AttributesFormatString=%<ID>
  Load Flow Bus15 : powerlib/Measurements/Load Flow Bus  LConnTagsString=a|b|c  RConnTagsString=a|b|c  Phases=ABC  Connectors=on both sides  ID=830  Vbase=Vnom  Vref=[0.9894 0.9982 0.9938]  Vangle=[-2.63 -123.39 117.25]  VLF=1  VLFb=1  VLFc=1  angleLF=0  angleLFb=0  angleLFc=0
      settings: AttributesFormatString=%<ID>
  Load Flow Bus16 : powerlib/Measurements/Load Flow Bus  LConnTagsString=a|b|c  RConnTagsString=a|b|c  Phases=ABC  Connectors=on both sides  ID=854  Vbase=Vnom  Vref=[0.989 0.9978 0.9934]  Vangle=[-2.64 -123.4 117.24]  VLF=1  VLFb=1  VLFc=1  angleLF=0  angleLFb=0  angleLFc=0
      settings: AttributesFormatString=%<ID>
  Load Flow Bus17 : powerlib/Measurements/Load Flow Bus  LConnTagsString=a  Phases=B  Connectors=on one side  ID=856  Vbase=Vnom  Vref=0.9977  Vangle=-123.41  VLF=1  VLFb=1  VLFc=1  angleLF=0  angleLFb=0  angleLFc=0
      settings: AttributesFormatString=%<ID>
  Load Flow Bus18 : powerlib/Measurements/Load Flow Bus  LConnTagsString=a|b|c  RConnTagsString=a|b|c  Phases=ABC  Connectors=on both sides  ID=852  Vbase=Vnom  Vref=[0.9581 0.968 0.9637]  Vangle=[-3.11 -124.18 116.33]  VLF=1  VLFb=1  VLFc=1  angleLF=0  angleLFb=0  angleLFc=0
      settings: AttributesFormatString=%<ID>
  Load Flow Bus19 : powerlib/Measurements/Load Flow Bus  LConnTagsString=a|b|c  RConnTagsString=a|b|c  Phases=ABC  Connectors=on both sides  ID=832  Vbase=Vnom  Vref=[1.0359 1.0345 1.036]  Vangle=[-3.11 -124.18 116.33]  VLF=1  VLFb=1  VLFc=1  angleLF=0  angleLFb=0  angleLFc=0
      settings: AttributesFormatString=%<ID>
  Load Flow Bus2 : powerlib/Measurements/Load Flow Bus  LConnTagsString=a|b|c  RConnTagsString=a|b|c  Phases=ABC  Connectors=on both sides  ID=806  Vbase=Vnom  Vref=[1.0457 1.0474 1.0474]  Vangle=[-0.08 -120.11 119.92]  VLF=1  VLFb=1  VLFc=1  angleLF=0  angleLFb=0  angleLFc=0
      settings: AttributesFormatString=%<ID>
  Load Flow Bus20 : powerlib/Measurements/Load Flow Bus  LConnTagsString=a|b|c  RConnTagsString=a|b|c  Phases=ABC  Connectors=on both sides  ID=888  Vbase=Vnom1  Vref=[0.9996 0.9983 1]  Vangle=[-4.64 -125.73 114.82]  VLF=1  VLFb=1  VLFc=1  angleLF=0  angleLFb=0  angleLFc=0
      settings: AttributesFormatString=%<ID>
  Load Flow Bus21 : powerlib/Measurements/Load Flow Bus  LConnTagsString=a|b|c  RConnTagsString=a|b|c  Phases=ABC  Connectors=on both sides  ID=890  Vbase=Vnom1  Vref=[0.9167 0.9235 0.9177]  Vangle=[-5.19 -126.78 113.98]  VLF=1  VLFb=1  VLFc=1  angleLF=0  angleLFb=0  angleLFc=0
      settings: AttributesFormatString=%<ID>
  Load Flow Bus22 : powerlib/Measurements/Load Flow Bus  LConnTagsString=a|b|c  RConnTagsString=a|b|c  Phases=ABC  Connectors=on both sides  ID=858  Vbase=Vnom  Vref=[1.0336 1.0322 1.0338]  Vangle=[-3.17 -124.28 116.22]  VLF=1  VLFb=1  VLFc=1  angleLF=0  angleLFb=0  angleLFc=0
      settings: AttributesFormatString=%<ID>
  Load Flow Bus23 : powerlib/Measurements/Load Flow Bus  LConnTagsString=a  Phases=A  Connectors=on one side  ID=864  Vbase=Vnom  Vref=1.0336  Vangle=-3.17  VLF=1  VLFb=1  VLFc=1  angleLF=0  angleLFb=0  angleLFc=0
      settings: AttributesFormatString=%<ID>
  Load Flow Bus24 : powerlib/Measurements/Load Flow Bus  LConnTagsString=a|b|c  RConnTagsString=a|b|c  Phases=ABC  Connectors=on both sides  ID=834  Vbase=Vnom  Vref=[1.0309 1.0295 1.0313]  Vangle=[-3.24 -124.39 116.09]  VLF=1  VLFb=1  VLFc=1  angleLF=0  angleLFb=0  angleLFc=0
      settings: AttributesFormatString=%<ID>
  Load Flow Bus25 : powerlib/Measurements/Load Flow Bus  LConnTagsString=a|b|c  RConnTagsString=a|b|c  Phases=ABC  Connectors=on both sides  ID=860  Vbase=Vnom  Vref=[1.0305 1.0291 1.031]  Vangle=[-3.24 -124.39 116.09]  VLF=1  VLFb=1  VLFc=1  angleLF=0  angleLFb=0  angleLFc=0
      settings: AttributesFormatString=%<ID>
  Load Flow Bus26 : powerlib/Measurements/Load Flow Bus  LConnTagsString=a|b|c  RConnTagsString=a|b|c  Phases=ABC  Connectors=on both sides  ID=836  Vbase=Vnom  Vref=[1.0303 1.0287 1.0308]  Vangle=[-3.23 -124.39 116.09]  VLF=1  VLFb=1  VLFc=1  angleLF=0  angleLFb=0  angleLFc=0
      settings: AttributesFormatString=%<ID>
  Load Flow Bus27 : powerlib/Measurements/Load Flow Bus  LConnTagsString=a|b|c  RConnTagsString=a|b|c  Phases=ABC  Connectors=on both sides  ID=840  Vbase=Vnom  Vref=[1.0303 1.0287 1.0308]  Vangle=[-3.23 -124.39 116.09]  VLF=1  VLFb=1  VLFc=1  angleLF=0  angleLFb=0  angleLFc=0
      settings: AttributesFormatString=%<ID>
  Load Flow Bus29 : powerlib/Measurements/Load Flow Bus  LConnTagsString=a  Phases=B  Connectors=on one side  ID=838  Vbase=Vnom  Vref=1.0285  Vangle=-124.39  VLF=1  VLFb=1  VLFc=1  angleLF=0  angleLFb=0  angleLFc=0
      settings: AttributesFormatString=%<ID>
  Load Flow Bus3 : powerlib/Measurements/Load Flow Bus  LConnTagsString=a|b|c  RConnTagsString=a|b|c  Phases=ABC  Connectors=on both sides  ID=808  Vbase=Vnom  Vref=[1.0136 1.0296 1.0289]  Vangle=[-0.75 -120.95 119.3]  VLF=1  VLFb=1  VLFc=1  angleLF=0  angleLFb=0  angleLFc=0
      settings: AttributesFormatString=%<ID>
  Load Flow Bus30 : powerlib/Measurements/Load Flow Bus  LConnTagsString=a|b|c  RConnTagsString=a|b|c  Phases=ABC  Connectors=on both sides  ID=842  Vbase=Vnom  Vref=[1.0309 1.0294 1.0313]  Vangle=[-3.25 -124.39 116.09]  VLF=1  VLFb=1  VLFc=1  angleLF=0  angleLFb=0  angleLFc=0
      settings: AttributesFormatString=%<ID>
  Load Flow Bus31 : powerlib/Measurements/Load Flow Bus  LConnTagsString=a|b|c  RConnTagsString=a|b|c  Phases=ABC  Connectors=on both sides  ID=844  Vbase=Vnom  Vref=[1.0307 1.0291 1.0311]  Vangle=[-3.27 -124.42 116.06]  VLF=1  VLFb=1  VLFc=1  angleLF=0  angleLFb=0  angleLFc=0
      settings: AttributesFormatString=%<ID>
  Load Flow Bus32 : powerlib/Measurements/Load Flow Bus  LConnTagsString=a|b|c  RConnTagsString=a|b|c  Phases=ABC  Connectors=on both sides  ID=846  Vbase=Vnom  Vref=[1.0309 1.0291 1.0313]  Vangle=[-3.32 -124.46 116.01]  VLF=1  VLFb=1  VLFc=1  angleLF=0  angleLFb=0  angleLFc=0
      settings: AttributesFormatString=%<ID>
  Load Flow Bus33 : powerlib/Measurements/Load Flow Bus  LConnTagsString=a|b|c  RConnTagsString=a|b|c  Phases=ABC  Connectors=on both sides  ID=848  Vbase=Vnom  Vref=[1.031 1.0291 1.0314]  Vangle=[-3.32 -124.47 116]  VLF=1  VLFb=1  VLFc=1  angleLF=0  angleLFb=0  angleLFc=0
      settings: AttributesFormatString=%<ID>
  Load Flow Bus34 : powerlib/Measurements/Load Flow Bus  LConnTagsString=a  Phases=A  Connectors=on one side  ID=open862  Vbase=Vnom  Vref=1.0303  Vangle=-3.23  VLF=1  VLFb=1  VLFc=1  angleLF=0  angleLFb=0  angleLFc=0
      settings: AttributesFormatString=%<ID>
  Load Flow Bus35 : powerlib/Measurements/Load Flow Bus  LConnTagsString=a  Phases=C  Connectors=on one side  ID=open862  Vbase=Vnom  Vref=1.0308  Vangle=116.09  VLF=1  VLFb=1  VLFc=1  angleLF=0  angleLFb=0  angleLFc=0
      settings: AttributesFormatString=%<ID>
  Load Flow Bus36 : powerlib/Measurements/Load Flow Bus  LConnTagsString=a  RConnTagsString=a  Phases=B  Connectors=on both sides  ID=862  Vbase=Vnom  Vref=1.0287  Vangle=-124.39  VLF=1  VLFb=1  VLFc=1  angleLF=0  angleLFb=0  angleLFc=0
      settings: AttributesFormatString=%<ID>
  Load Flow Bus4 : powerlib/Measurements/Load Flow Bus  LConnTagsString=a|b|c  RConnTagsString=a|b|c  Phases=ABC  Connectors=on both sides  ID=812  Vbase=Vnom  Vref=[0.9763 1.01 1.0069]  Vangle=[-1.57 -121.92 118.59]  VLF=1  VLFb=1  VLFc=1  angleLF=0  angleLFb=0  angleLFc=0
      settings: AttributesFormatString=%<ID>
  Load Flow Bus5 : powerlib/Measurements/Load Flow Bus  LConnTagsString=a|b|c  RConnTagsString=a|b|c  Phases=ABC  Connectors=on both sides  ID=814  Vbase=Vnom  Vref=[0.9467 0.9945 0.9893]  Vangle=[-2.26 -122.7 118.01]  VLF=1  VLFb=1  VLFc=1  angleLF=0  angleLFb=0  angleLFc=0
      settings: AttributesFormatString=%<ID>
  Load Flow Bus6 : powerlib/Measurements/Load Flow Bus  LConnTagsString=a  Phases=B  Connectors=on one side  ID=810  Vbase=Vnom  Vref=1.0294  Vangle=-120.95  VLF=1  VLFb=1  VLFc=1  angleLF=0  angleLFb=0  angleLFc=0
      settings: AttributesFormatString=%<ID>
  Load Flow Bus7 : powerlib/Measurements/Load Flow Bus  LConnTagsString=a|b|c  RConnTagsString=a|b|c  Phases=ABC  Connectors=on both sides  ID=850  Vbase=Vnom  Vref=[1.0176 1.0255 1.0203]  Vangle=[-2.26 -122.7 118.01]  VLF=1  VLFb=1  VLFc=1  angleLF=0  angleLFb=0  angleLFc=0
      settings: AttributesFormatString=%<ID>
  Load Flow Bus8 : powerlib/Measurements/Load Flow Bus  LConnTagsString=a|b|c  RConnTagsString=a|b|c  Phases=ABC  Connectors=on both sides  ID=816  Vbase=Vnom  Vref=[1.0172 1.0253 1.02]  Vangle=[-2.26 -122.71 1.02]  VLF=1  VLFb=1  VLFc=1  angleLF=0  angleLFb=0  angleLFc=0
      settings: AttributesFormatString=%<ID>
  Load Flow Bus9 : powerlib/Measurements/Load Flow Bus  LConnTagsString=a|b|c  RConnTagsString=a|b|c  Phases=ABC  Connectors=on both sides  ID=824  Vbase=Vnom  Vref=[1.0082 1.0158 1.0116]  Vangle=[-2.37 -122.94 117.76]  VLF=1  VLFb=1  VLFc=1  angleLF=0  angleLFb=0  angleLFc=0
      settings: AttributesFormatString=%<ID>
  MultiStateImage : MultiStateImageBlock  ScaleMode=Fill
  Power-Flow : Subsystem
      mask Display: disp('Power-Flow\nResults')
  XF-10 24.9kV / 4.16kV : powerlib/Elements/Three-Phase Transformer (Two Windings)  Winding1Connection=Yg  Winding2Connection=Yg  CoreType=Three single-phase transformers  SetSaturation=off  Hysteresis=off  DataFile='hysteresis'  SetInitialFlux=off  Measurements=None  UNITS=pu  NominalPower=[ 500e3 , 60 ]  Winding1=[ 24.9e3 , 0.019 , 0.0408 ]  Winding2=[ 4.16e3 , 0 , 0 ]  Rm=500  Lm=500  L0=0.5  Saturation=[ 0,0 ; 0.0024,1.2 ; 1.0,1.52 ]  InitialFluxes=[ 0.8 , -0.8 , 0.7 ]  BreakLoop=off  DiscreteSolver=Trapezoidal iterative  DataType=off  TransfoNumber=1
  powergui : powerlib/powergui  Priority=1  SimulationMode=Phasor  SampleTime=50e-6  frequency=60  Iterations=50  frequencyindice=60  Pbase=100e3  ErrMax=0.0001  UnitsV=kV  UnitsW=kW  buscounter=0  FunctionMessages=off  echomessages=off  EnableUseOfTLC=off  CurrentSourceSwitches=off  DisableSnubberDevices=off  DisableRonSwitches=off  DisableVfSwitches=off  DisplayEquations=off  AutomaticDiscreteSolvers=off  SolverType=Tustin/Backward Euler (TBE)  Interpol=off  ExternalGateDelay=off  methode=off  Ts=100  x0status=blocks  SPID=off  SwTol=0  HookPort=off  NonlinearTolerance=1e-4  nMaxIteration=100  ContinueOnMaxIteration=off  RestoreLinks=warning  ResistiveCurrentMeasurement=off  Frange=[0:2:500]  Ylog=off  Xlog=on  ShowGrid=off  save=off  variable=ZData  structure=0  ZoomFFT=on  StartTime=0.0  cycles=1  DisplayStyle=1  fundamental=60  FreqAxis=off  MaxFrequency=1000  frequencyindicesteady=1  RmsSteady=1  display=off
  wires:
  Constant3/1 -> Breaker832-858/1
  Constant5/1 -> Breaker836-862/1
  Constant4/1 -> Breaker834-842/1
  Constant1/1 -> Breaker850-816/1
  Constant2/1 -> Breaker818-820/1
  connections:
  800-802/RConn1 -- Load Flow Bus1/LConn1
  800-802/RConn2 -- Load Flow Bus1/LConn2
  800-802/RConn3 -- Load Flow Bus1/LConn3
  802/LConn1 -- Load Flow Bus1/RConn1
  802/LConn2 -- Load Flow Bus1/RConn2
  802/LConn3 -- Load Flow Bus1/RConn3
  802-806/LConn1 -- 802/RConn1 -- 802 Yg PQ/LConn1
  802-806/LConn2 -- 802/RConn2 -- 802 Yg PQ/LConn2
  802-806/LConn3 -- 802/RConn3 -- 802 Yg PQ/LConn3
  Load Flow Bus2/LConn1 -- 802-806/RConn1 -- 806 Yg PQ/LConn1
  Load Flow Bus2/LConn2 -- 802-806/RConn2 -- 806 Yg PQ/LConn2
  Load Flow Bus2/LConn3 -- 806 Yg PQ/LConn3 -- 802-806/RConn3
  808/LConn2 -- Load Flow Bus3/RConn2
  808/LConn3 -- Load Flow Bus3/RConn3
  Load Flow Bus3/LConn3 -- 806-808/RConn3
  Load Flow Bus3/LConn1 -- 806-808/RConn1
  Load Flow Bus3/LConn2 -- 806-808/RConn2
  808/LConn1 -- Load Flow Bus3/RConn1
  Load Flow Bus4/LConn3 -- 808-812/RConn3
  Load Flow Bus4/LConn1 -- 808-812/RConn1
  Load Flow Bus4/LConn2 -- 808-812/RConn2
  808-812/LConn1 -- 808/RConn1
  808-812/LConn2 -- 808 Y-I/LConn1 -- 808-810/LConn1 -- 808/RConn2
  808-812/LConn3 -- 808/RConn3
  Load Flow Bus5/LConn3 -- 812-814/RConn3
  Load Flow Bus5/LConn1 -- 812-814/RConn1
  Load Flow Bus5/LConn2 -- 812-814/RConn2
  Load Flow Bus7/LConn1 -- 814-850/RConn1
  Load Flow Bus7/LConn2 -- 814-850/RConn2
  Load Flow Bus7/LConn3 -- 814-850/RConn3
  816/LConn3 -- Load Flow Bus8/RConn3
  816/LConn1 -- Load Flow Bus8/RConn1
  816/LConn2 -- Load Flow Bus8/RConn2
  Load Flow Bus8/LConn2 -- 850-816/RConn2
  Load Flow Bus8/LConn3 -- 850-816/RConn3
  Load Flow Bus8/LConn1 -- 850-816/RConn1
  Load Flow Bus9/LConn2 -- 824 D-I/LConn2 -- 816-824/RConn2
  824/LConn1 -- Load Flow Bus9/RConn1
  Load Flow Bus9/LConn1 -- 824 D-I/LConn1 -- 816-824/RConn1
  824/LConn2 -- Load Flow Bus9/RConn2
  824/LConn3 -- Load Flow Bus9/RConn3
  Load Flow Bus9/LConn3 -- 824 D-I/LConn3 -- 816-824/RConn3
  816-824/LConn1 -- 816-818/LConn1 -- 816 D-I/LConn1 -- 816/RConn1
  816-824/LConn2 -- 816 D-I/LConn2 -- 816/RConn2
  816-824/LConn3 -- 816 D-I/LConn3 -- 816/RConn3
  824-828/LConn1 -- 824 Y-PQ/LConn1 -- 824/RConn1
  824-828/LConn2 -- 824 Y-PQ/LConn2 -- 824-826/LConn1 -- 824 Y-I/LConn1 -- 824/RConn2
  824-828/LConn3 -- 824 Y-PQ/LConn3 -- 824/RConn3
  818-820/LConn1 -- Breaker818-820/RConn1 -- 818 Y-Z/LConn1
  820-822/LConn1 -- 820/RConn1 -- 820 Y-PQ/LConn1
  820 Y-Z/LConn1 -- 818-820/RConn1 -- Load Flow Bus12/LConn1
  822 Y-PQ/LConn1 -- 822/RConn1 -- Load Flow Bus13/LConn1
  828/LConn2 -- Load Flow Bus14/RConn2
  Load Flow Bus14/LConn3 -- 824-828/RConn3 -- 828 Y-PQ/LConn3
  828/LConn1 -- Load Flow Bus14/RConn1
  Load Flow Bus14/LConn1 -- 828 Y-PQ/LConn1 -- 824-828/RConn1
  828/LConn3 -- Load Flow Bus14/RConn3
  Load Flow Bus14/LConn2 -- 824-828/RConn2 -- 828 Y-PQ/LConn2
  830 Y-PQ/LConn1 -- Load Flow Bus15/LConn1 -- 828-830/RConn1
  830 Y-PQ/LConn2 -- Load Flow Bus15/LConn2 -- 828-830/RConn2
  830 Y-PQ/LConn3 -- Load Flow Bus15/LConn3 -- 828-830/RConn3
  828-830/LConn1 -- 828 Y-PQ1/LConn1 -- 828/RConn1
  828-830/LConn2 -- 828 Y-PQ1/LConn2 -- 828/RConn2
  828-830/LConn3 -- 828 Y-PQ1/LConn3 -- 828/RConn3
  Load Flow Bus16/LConn1 -- 830-854/RConn1
  Load Flow Bus16/LConn2 -- 830-854/RConn2
  Load Flow Bus16/LConn3 -- 830-854/RConn3
  Load Flow Bus18/LConn1 -- 854-852/RConn1
  Load Flow Bus18/LConn3 -- 854-852/RConn3
  Load Flow Bus18/LConn2 -- 854-852/RConn2
  Load Flow Bus19/LConn3 -- 852-832/RConn3
  Load Flow Bus19/LConn2 -- 852-832/RConn2
  832/LConn1 -- Load Flow Bus19/RConn1
  Load Flow Bus19/LConn1 -- 852-832/RConn1
  832/LConn2 -- Load Flow Bus19/RConn2
  832/LConn3 -- Load Flow Bus19/RConn3
  854-856/LConn1 -- 854 Y-PQ/LConn1 -- 854-852/LConn2 -- 854/RConn2
  890/LConn1 -- Load Flow Bus21/RConn1
  890/LConn2 -- Load Flow Bus21/RConn2
  Load Flow Bus21/LConn1 -- 888-890/RConn1
  Load Flow Bus21/LConn2 -- 888-890/RConn2
  890/LConn3 -- Load Flow Bus21/RConn3
  Load Flow Bus21/LConn3 -- 888-890/RConn3
  890 D-I/LConn1 -- 890/RConn1
  890 D-I/LConn2 -- 890/RConn2
  890 D-I/LConn3 -- 890/RConn3
  858-834/LConn2 -- 858 D-PQ/LConn2 -- 858/RConn2
  Load Flow Bus22/LConn3 -- 858 D-Z/LConn3 -- 832-858/RConn3
  Load Flow Bus22/LConn1 -- 858 D-Z/LConn1 -- 832-858/RConn1
  858/LConn3 -- Load Flow Bus22/RConn3
  Load Flow Bus22/LConn2 -- 858 D-Z/LConn2 -- 832-858/RConn2
  858/LConn1 -- Load Flow Bus22/RConn1
  858-834/LConn1 -- 858 D-PQ/LConn1 -- 858-864/LConn1 -- 858 Y-PQ/LConn1 -- 858/RConn1
  858/LConn2 -- Load Flow Bus22/RConn2
  858-834/LConn3 -- 858 D-PQ/LConn3 -- 858/RConn3
  Load Flow Bus25/LConn3 -- 860 D-Z/LConn3 -- 834-860/RConn3
  834-860/LConn1 -- 834 D-Z/LConn1 -- Breaker834-842/RConn1 -- 834/RConn1
  834/LConn2 -- Load Flow Bus24/RConn2
  860/LConn3 -- Load Flow Bus25/RConn3
  834/LConn3 -- Load Flow Bus24/RConn3
  860/LConn1 -- Load Flow Bus25/RConn1
  Load Flow Bus24/LConn2 -- 834 D-PQ/LConn2 -- 858-834/RConn2
  Load Flow Bus24/LConn1 -- 834 D-PQ/LConn1 -- 858-834/RConn1
  Load Flow Bus24/LConn3 -- 834 D-PQ/LConn3 -- 858-834/RConn3
  834/LConn1 -- Load Flow Bus24/RConn1
  Load Flow Bus25/LConn2 -- 860 D-Z/LConn2 -- 834-860/RConn2
  860/LConn2 -- Load Flow Bus25/RConn2
  834-860/LConn3 -- 834 D-Z/LConn3 -- Breaker834-842/RConn3 -- 834/RConn3
  834-860/LConn2 -- 834 D-Z/LConn2 -- Breaker834-842/RConn2 -- 834/RConn2
  Load Flow Bus25/LConn1 -- 860 D-Z/LConn1 -- 834-860/RConn1
  XF-10 24.9kV / 4.16kV/LConn1 -- 832/RConn1 -- Breaker832-858/RConn1
  XF-10 24.9kV / 4.16kV/LConn2 -- 832/RConn2 -- Breaker832-858/RConn2
  832 D-Z/LConn3 -- 832-858/LConn3 -- Breaker832-858/LConn3
  Load Flow Bus26/LConn1 -- 836 D-PQ/LConn1 -- 860-836/RConn1
  Load Flow Bus26/LConn2 -- 836 D-PQ/LConn2 -- 860-836/RConn2
  836/LConn3 -- Load Flow Bus26/RConn3
  836/LConn1 -- Load Flow Bus26/RConn1
  Load Flow Bus26/LConn3 -- 836 D-PQ/LConn3 -- 860-836/RConn3
  836/LConn2 -- Load Flow Bus26/RConn2
  860-836/LConn1 -- 860 D-PQ/LConn1 -- 860 Y-PQ/LConn1 -- 860/RConn1
  860-836/LConn2 -- 860 D-PQ/LConn2 -- 860 Y-PQ/LConn2 -- 860/RConn2
  860-836/LConn3 -- 860 D-PQ/LConn3 -- 860 Y-PQ/LConn3 -- 860/RConn3
  Load Flow Bus27/LConn1 -- 836-840/RConn1 -- 840 D-I/LConn1
  Load Flow Bus27/LConn2 -- 836-840/RConn2 -- 840 D-I/LConn2
  840/LConn1 -- Load Flow Bus27/RConn1
  840/LConn2 -- Load Flow Bus27/RConn2
  Load Flow Bus27/LConn3 -- 836-840/RConn3 -- 840 D-I/LConn3
  840/LConn3 -- Load Flow Bus27/RConn3
  836-840/LConn1 -- Breaker836-862/LConn1 -- 836/RConn1 -- 836 D-I/LConn1
  836-840/LConn2 -- Breaker836-862/LConn2 -- 836/RConn2 -- 836 D-I/LConn2
  836-840/LConn3 -- Breaker836-862/LConn3 -- 836/RConn3 -- 836 D-I/LConn3
  840 Y-I/LConn1 -- 840/RConn1
  840 Y-I/LConn2 -- 840/RConn2
  840 Y-I/LConn3 -- 840/RConn3
  Load Flow Bus30/LConn1 -- 834-842/RConn1
  842/LConn2 -- Load Flow Bus30/RConn2
  842/LConn3 -- Load Flow Bus30/RConn3
  Load Flow Bus30/LConn2 -- 834-842/RConn2
  Load Flow Bus30/LConn3 -- 834-842/RConn3
  842/LConn1 -- Load Flow Bus30/RConn1
  Load Flow Bus31/LConn2 -- 844 Y-PQ/LConn2 -- 842-844/RConn2
  844/LConn2 -- Load Flow Bus31/RConn2
  Load Flow Bus31/LConn1 -- 844 Y-PQ/LConn1 -- 842-844/RConn1
  844/LConn1 -- Load Flow Bus31/RConn1
  842-844/LConn1 -- 842 Y-PQ/LConn1 -- 842/RConn1
  842-844/LConn2 -- 842 Y-PQ/LConn2 -- 842/RConn2
  842-844/LConn3 -- 842 Y-PQ/LConn3 -- 842/RConn3
  Load Flow Bus32/LConn2 -- 844-846/RConn2 -- 846 Y-PQ/LConn2
  846/LConn2 -- Load Flow Bus32/RConn2
  Load Flow Bus32/LConn1 -- 844-846/RConn1 -- 846 Y-PQ/LConn1
  846/LConn1 -- Load Flow Bus32/RConn1
  844-846/LConn1 -- 844 Y-PQ1/LConn1 -- 844 Y-Z1/LConn1 -- 844 Y-Z/LConn1 -- 844/RConn1
  844-846/LConn2 -- 844 Y-PQ1/LConn2 -- 844 Y-Z1/LConn2 -- 844 Y-Z/LConn2 -- 844/RConn2
  844-846/LConn3 -- 844 Y-PQ1/LConn3 -- 844 Y-Z1/LConn3 -- 844 Y-Z/LConn3 -- 844/RConn3
  Load Flow Bus33/LConn2 -- 848 Y-PQ/LConn2 -- 846-848/RConn2
  848/LConn2 -- Load Flow Bus33/RConn2
  Load Flow Bus33/LConn1 -- 848 Y-PQ/LConn1 -- 846-848/RConn1
  848/LConn1 -- Load Flow Bus33/RConn1
  846-848/LConn1 -- 846 Y-PQ1/LConn1 -- 846/RConn1
  846-848/LConn2 -- 846 Y-PQ1/LConn2 -- 846/RConn2
  846-848/LConn3 -- 846 Y-PQ1/LConn3 -- 846/RConn3
  848 D-PQ/LConn1 -- 848 D-Z/LConn1 -- 848/RConn1
  848 D-PQ/LConn2 -- 848 D-Z/LConn2 -- 848/RConn2
  848 D-PQ/LConn3 -- 848 D-Z/LConn3 -- 848/RConn3
  Load Flow Bus20/LConn1 -- XF-10 24.9kV / 4.16kV/RConn1
  Load Flow Bus20/LConn2 -- XF-10 24.9kV / 4.16kV/RConn2
  Load Flow Bus20/LConn3 -- XF-10 24.9kV / 4.16kV/RConn3
  826 Y-I/LConn1 -- 826/RConn2 -- Load Flow Bus10/LConn1
  856 Y-PQ/LConn1 -- 856/RConn2 -- Load Flow Bus17/LConn1
  838 Y-PQ/LConn1 -- 838/RConn2 -- Load Flow Bus29/LConn1
  Ground1/LConn1 -- 810 Y-I/RConn1
  Ground2/LConn1 -- 818 Y-Z/RConn1
  Ground3/LConn1 -- 820 Y-Z/RConn1
  Ground4/LConn1 -- 820 Y-PQ/RConn1
  Ground5/LConn1 -- 822 Y-PQ/RConn1
  862-838/LConn1 -- 862 Y-PQ/LConn1 -- Load Flow Bus36/RConn1
  Ground8/LConn1 -- 824 Y-I/RConn1
  Ground9/LConn1 -- 826 Y-I/RConn1
  842-844/RConn3 -- 844 Y-PQ/LConn3 -- Load Flow Bus31/LConn3
  Load Flow Bus31/RConn3 -- 844/LConn3
  844-846/RConn3 -- 846 Y-PQ/LConn3 -- Load Flow Bus32/LConn3
  Load Flow Bus32/RConn3 -- 846/LConn3
  846-848/RConn3 -- 848 Y-PQ/LConn3 -- Load Flow Bus33/LConn3
  Load Flow Bus33/RConn3 -- 848/LConn3
  Ground10/LConn1 -- 854 Y-PQ/RConn1
  Ground11/LConn1 -- 856 Y-PQ/RConn1
  Ground12/LConn1 -- 858 Y-PQ/RConn1
  Ground13/LConn1 -- 864 Y-PQ/RConn1
  864 Y-PQ/LConn1 -- 864/RConn1 -- Load Flow Bus23/LConn1
  Ground14/LConn1 -- 862 Y-PQ/RConn1
  Ground15/LConn1 -- 838 Y-PQ/RConn1
  Load Flow Bus/RConn1 -- 800-802/LConn1
  Load Flow Bus/RConn2 -- 800-802/LConn2
  Load Flow Bus/RConn3 -- 800-802/LConn3
  830/LConn1 -- Load Flow Bus15/RConn1
  830/LConn2 -- Load Flow Bus15/RConn2
  830/LConn3 -- Load Flow Bus15/RConn3
  830-854/LConn1 -- 830 D-Z/LConn1 -- 830/RConn1
  830-854/LConn2 -- 830 D-Z/LConn2 -- 830/RConn2
  830-854/LConn3 -- 830 D-Z/LConn3 -- 830/RConn3
  810/LConn2 -- 808-810/RConn1
  816-818/RConn1 -- Load Flow Bus11/LConn1
  832 D-Z/LConn1 -- 832-858/LConn1 -- Breaker832-858/LConn1
  XF-10 24.9kV / 4.16kV/LConn3 -- Breaker832-858/RConn3 -- 832/RConn3
  832 D-Z/LConn2 -- 832-858/LConn2 -- Breaker832-858/LConn2
  Ground/LConn1 -- 808 Y-I/RConn1
  Breaker836-862/RConn1 -- 836-862/LConn1
  Breaker836-862/RConn2 -- 836-862/LConn2
  Breaker836-862/RConn3 -- 836-862/LConn3
  834-842/LConn1 -- Breaker834-842/LConn1
  834-842/LConn2 -- Breaker834-842/LConn2
  834-842/LConn3 -- Breaker834-842/LConn3
  Breaker850-816/LConn3 -- 850-816/LConn1
  Breaker850-816/LConn2 -- 850-816/LConn2
  Breaker850-816/LConn1 -- 850-816/LConn3
  818/LConn1 -- Load Flow Bus11/RConn1
  818/RConn1 -- Breaker818-820/LConn1
  818/RConn2 -- 818/RConn3 -- 818/LConn3 -- 818/LConn2 -- Ground6/LConn1
  806/RConn1 -- 806-808/LConn1
  806/LConn1 -- Load Flow Bus2/RConn1
  806/LConn2 -- Load Flow Bus2/RConn2
  806/RConn2 -- 806-808/LConn2
  806/RConn3 -- 806-808/LConn3
  806/LConn3 -- Load Flow Bus2/RConn3
  812/RConn1 -- 812-814/LConn1
  812/LConn1 -- Load Flow Bus4/RConn1
  812/LConn2 -- Load Flow Bus4/RConn2
  812/RConn2 -- 812-814/LConn2
  812/LConn3 -- Load Flow Bus4/RConn3
  812/RConn3 -- 812-814/LConn3
  814/RConn1 -- 814-850/LConn1
  814/LConn1 -- Load Flow Bus5/RConn1
  Load Flow Bus5/RConn2 -- 814/LConn2
  Load Flow Bus5/RConn3 -- 814/LConn3
  814/RConn2 -- 814-850/LConn2
  814-850/LConn3 -- 814/RConn3
  810/RConn3 -- 810/LConn1 -- 810/LConn3 -- Ground7/LConn1 -- 810/RConn1
  810/RConn2 -- 810 Y-I/LConn1 -- Load Flow Bus6/LConn1
  850/RConn1 -- Breaker850-816/RConn3
  850/RConn2 -- Breaker850-816/RConn2
  850/RConn3 -- Breaker850-816/RConn1
  850/LConn1 -- Load Flow Bus7/RConn1
  850/LConn2 -- Load Flow Bus7/RConn2
  850/LConn3 -- Load Flow Bus7/RConn3
  820/RConn2 -- 820/LConn3 -- 820/LConn2 -- Ground16/LConn1 -- 820/RConn3
  Load Flow Bus12/RConn1 -- 820/LConn1
  822/RConn2 -- 822/LConn3 -- 822/LConn2 -- Ground17/LConn1 -- 822/RConn3
  822/LConn1 -- 820-822/RConn1
  826/RConn3 -- 826/LConn1 -- 826/LConn3 -- Ground18/LConn1 -- 826/RConn1
  826/LConn2 -- 824-826/RConn1
  854/LConn1 -- Load Flow Bus16/RConn1
  854/LConn2 -- Load Flow Bus16/RConn2
  854/LConn3 -- Load Flow Bus16/RConn3
  854/RConn3 -- 854-852/LConn3
  854/RConn1 -- 854-852/LConn1
  Ground19/LConn1 -- 856/RConn1 -- 856/RConn3 -- 856/LConn1 -- 856/LConn3
  856/LConn2 -- 854-856/RConn1
  852/LConn1 -- Load Flow Bus18/RConn1
  852/LConn2 -- Load Flow Bus18/RConn2
  852/LConn3 -- Load Flow Bus18/RConn3
  852/RConn1 -- 852-832/LConn1
  852/RConn2 -- 852-832/LConn2
  852/RConn3 -- 852-832/LConn3
  888/LConn1 -- Load Flow Bus20/RConn1
  888/LConn2 -- Load Flow Bus20/RConn2
  888/LConn3 -- Load Flow Bus20/RConn3
  888/RConn1 -- 888-890/LConn1
  888/RConn2 -- 888-890/LConn2
  888/RConn3 -- 888-890/LConn3
  864/RConn3 -- 864/LConn2 -- 864/LConn3 -- Ground20/LConn1 -- 864/RConn2
  864/LConn1 -- 858-864/RConn1
  836-862/RConn1 -- 862/LConn1
  836-862/RConn2 -- 862/LConn2
  836-862/RConn3 -- 862/LConn3
  Load Flow Bus34/LConn1 -- 862/RConn1
  Load Flow Bus36/LConn1 -- 862/RConn2
  Load Flow Bus35/LConn1 -- 862/RConn3
  838/LConn3 -- 838/LConn1 -- 838/RConn1 -- 838/RConn3 -- Ground21/LConn1
  838/LConn2 -- 862-838/RConn1
  800 gen/RConn1 -- Load Flow Bus/LConn1
  800 gen/RConn2 -- Load Flow Bus/LConn2
  800 gen/RConn3 -- Load Flow Bus/LConn3
